simulink model "FeedBack_Linearization"  (R2021b)
(part 8 of 9)

et1504 = ((t3141.*(t8.*(t92-t663)+t15.*(t621-t864))+t2289.*t3617+t2330.*t3620+t2627.*t3444+(t651-t1053).*(t958-t2263+dq7.*t1601+t15.*(t642+t896-t1137-t2220))-t2576.*(t987+t1806+t2261-t3154+t15.*t948)).*(et1333+et1334))./2.0-(t3789.*(et1335+et1336+et1337+et1338+et1339+et1340+et1341+et1342+et1343+et1344))./2.0;
et1505 = t3784.*(t70.*1.8866e-1+t612.*1.8866e-1-t6.*(t88-t617).*5.000000000000001e-5-t13.*(t88-t617).*2.37e-3).*(3.41e+2./1.0e+2);
et1506 = ((t2817+t3324+t3433.*(t614+t13.*(t86-t652))+t2832.*(t639-t1128-t2181+dq5.*t13.*(t86-t652))+t2974.*(t92-t663)+t3422.*(t653-t838)).*(et1345+et1346+et1347+et1348))./2.0-(t3826.*(t609+t846+t847))./2.0+et1349.*et1350-((t3163.*(t8.*(t92-t663)+t15.*(t621-t864))-t1697.*t3336-t2315.*t3618-t2576.*t3437+t2627.*(t933+t1888+t2483+t8.*(t932+t942+t2215+t7.*(t882-t2179)))+t3619.*(t908+t15.*(t921+t14.*(t86-t652)))).*(et1351+et1352))./2.0+(t3060.*(et1353+et1354+et1355+et1356))./2.0-((t859-t1791+t1066.*(t86-t652)).*(et1357+et1358+et1359))./2.0;
et1507 = t3798.*(et1360+et1361+et1362).*(-3.5432e-1)+et1363.*et1364+t3776.*(et1365+et1366).*3.38795-((t3429.*(t1386+t7.*(t88-t617))-t1207.*t3159+t2315.*t3312-(t908+t15.*(t921+t14.*(t86-t652))).*(t884+t1578-t2180+t14.*(t639-t1128-t2181+dq5.*t13.*(t86-t652)))-t1697.*(t631-t885+t1132-t2224)+t2074.*(t926+t988+t1886+t2207+t15.*(-t928+t984+t992+t2187+t2240))).*(et1367+et1368))./2.0;
et1508 = t3674.*(t235+t349+t456+t457+t512+t697.*4.9e-4-t705.*2.019e-2+t1213.*4.9e-4-t1219.*2.019e-2+t1667+t1702+t1710+t1718+t1720+t2072+t2111+t2125).*3.38795;
et1509 = et1369.*et1370-((t6.*(t88-t617).*(t653-t838)-t6.*t831.*(t614+t13.*(t86-t652))+t6.*t573.*(t92-t663)).*(et1371+et1372+et1373))./2.0+et1374.*et1375+(t3824.*(t604.*t815-t572.*(t86-t652)+t10.*t11.*t606))./2.0+(et1376+et1377).*(et1378+et1379+et1380).*3.5432e-1-(t3060.*(et1381+et1382+et1383+et1384+et1385))./2.0+(t3839.*(et1386+et1387+et1388+et1389+et1390))./2.0-((t2735.*(t1529+t15.*(t92-t663))-t1700.*t3618-t1776.*t3619-t2601.*t3161+t3336.*(t648-t657)+t2654.*(t927-t935-t2183+t2206+dq6.*t14.*(t86-t652))).*(et1391+et1392))./2.0+(t3828.*(et1393+et1394+et1395+et1396+et1397))./2.0;
et1510 = (t3840.*(t2074.*(t921+t14.*(t86-t652))+t1738.*(t1386+t7.*(t88-t617))+t1024.*t1207))./2.0-(t3610.*(et1398+et1399+et1400+et1401+et1402+et1403+et1404+et1405+et1406+et1407+et1408))./2.0+(t3610.*(et1409+et1410+et1411+et1412+et1413+et1414+et1415+et1416+et1417))./2.0-(t3666.*(et1418+et1419+et1420))./2.0+((t606.*t827+t815.*t1206-t1295.*(t86-t652)).*(et1421+et1422+et1423))./2.0+et1424.*et1425+(t3842.*(t13.*t831.*t2035+t13.*t573.*(t621-t864)-t13.*t2000.*(t88-t617)))./2.0-t3823.*(et1426+et1427).*3.38795;
et1511 = ((t3140+t3489+t3720+t2832.*(t884+t1578-t2180+t14.*(t639-t1128-t2181+dq5.*t13.*(t86-t652)))+t3436.*(t92-t663)+t3685.*(t653-t838)).*(et1428+et1429+et1430+et1431+et1432))./2.0-t3821.*(et1433+et1434).*3.5432e-1-((-t2961+t3358+t3312.*(t653-t838)).*(et1435+et1436+et1437+et1438+et1439+et1440+et1441+et1442+et1443))./2.0-(t3782.*(et1444+et1445+et1446+et1447+et1448+et1449+et1450+et1451+et1452))./2.0+(t3192.*(et1453+et1454+et1455+et1456+et1457))./2.0;
et1512 = ((t1700.*t2816+t1776.*t2832-(t614+t13.*(t86-t652)).*(t927-t935-t2183+t2206+dq6.*t14.*(t86-t652))-t2735.*(t92-t663)-t2196.*(t648-t657)+t3161.*(t653-t838)).*(et1458+et1459))./2.0-((t3377+t2074.*(t878-t1582+t2184+t7.*(t639-t1128-t2181+dq5.*t13.*(t86-t652)))+t1207.*(t642+t896-t1137-t2220)).*(et1460+et1461+et1462+et1463+et1464+et1465+et1466+et1467+et1468))./2.0;
et1513 = (t2601.*(t853+t983+t2264+t2503)+t2330.*(t884+t1578-t2180+t14.*(t639-t1128-t2181+dq5.*t13.*(t86-t652)))+t2289.*t3312+t2654.*t3168+(t1529+t15.*(t92-t663)).*(t673+t692-t1123-t1805)+(t651-t1053).*(t631-t885+t1132-t2224)).*(et1469+et1470).*(-1.0./2.0)+(t3782.*(et1471+et1472+et1473+et1474+et1475+et1476+et1477+et1478+et1479+et1480))./2.0;
et1514 = t3679.*(t30.*2.0e-4+t33.*5.267999999999999e-2-t82.*5.267999999999999e-2+t89.*2.0e-4).*2.61155;
et1515 = t3780.*(t70.*5.267999999999999e-2+t88.*2.0e-4+t612.*5.267999999999999e-2-t617.*2.0e-4).*(-2.61155);
et1516 = t3781.*(t79.*2.0e-4+t86.*5.267999999999999e-2-t652.*5.267999999999999e-2+t660.*2.0e-4).*(-2.61155);
et1517 = (t1843+t2621+t2648+t606.*t2165+t815.*t2828-(t86-t652).*(t639-t1128-t2181+dq5.*t13.*(t86-t652))).*(et1481+et1482).*(-1.0./2.0)+((t3502+t3544-t3547+t2972.*(t621-t864)+t2196.*(t642+t896-t1137-t2220)+t2816.*(t1487+t2219-t2864+dq6.*t7.*(t88-t617))).*(et1483+et1484+et1485+et1486+et1487))./2.0+et1488.*et1489;
et1518 = -t3291+t3365.*2.900000000000001e-4+t3527+t3642+t3654-t3662-t3665+t2654.*(t884+t1578-t2180+t14.*(t639-t1128-t2181+dq5.*t13.*(t86-t652))).*2.9e-4;
et1519 = t3336.*(t8.*(t92-t663)+t15.*(t621-t864)).*2.94e-3;
et1520 = t2942+t3260+t3261-t1295.*(t878-t1582+t2184+t7.*(t639-t1128-t2181+dq5.*t13.*(t86-t652))).*5.0e-5+t1625.*(t1386+t7.*(t88-t617)).*3.0e-5;
et1521 = t2861.*(t614+t13.*(t86-t652)).*(-1.000000000000001e-3)+t2823.*(t1386+t7.*(t88-t617)).*3.0e-5;
et1522 = t994.*t1207.*3.0e-5+t7.*t3171-t7.*t3358.*3.0e-5+t7.*t3388;
et1523 = t1207.*t2262.*3.0e-5-t1661.*t2074.*3.0e-5;
et1524 = t2074.*t2857.*(-3.0e-5)-t2266.*(t92-t663).*1.000000000000001e-3;
et1525 = t2825.*(t653-t838).*(-1.000000000000001e-3)+t827.*(t642+t896-t1137-t2220).*5.0e-5;
et1526 = t1206.*(t1487+t2219-t2864+dq6.*t7.*(t88-t617)).*5.0e-5+dq6.*t7.*t876.*5.000000000000004e-4;
et1527 = dq6.*t7.*t1462.*5.000000000000004e-4+dq6.*t7.*t1574.*5.000000000000004e-4;
et1528 = -t3294+t3365.*7.950000000000001e-3+t3528+t3648+t3658-t3660-t3663+t2654.*(t884+t1578-t2180+t14.*(t639-t1128-t2181+dq5.*t13.*(t86-t652))).*2.2e-4;
et1529 = t3336.*(t8.*(t92-t663)+t15.*(t621-t864)).*2.900000000000001e-4;
et1530 = t1516.*2.324e-2+t1528.*3.466000000000001e-2+t1668.*2.324e-2+t14.*(t614+t13.*(t86-t652)).*1.9738e-1;
et1531 = t7.*t8.*(t614+t13.*(t86-t652)).*(-3.466000000000001e-2);
et1532 = t2363.*(t1386+t7.*(t88-t617)).*(-7.950000000000001e-3)+t1779.*(t8.*(t92-t663)+t15.*(t621-t864)).*2.900000000000001e-4;
et1533 = t1207.*t1811.*(-7.950000000000001e-3)+t2074.*t2380.*7.950000000000001e-3;
et1534 = t2352.*t2576.*(-2.900000000000001e-4)-t2374.*t2627.*2.900000000000001e-4;
et1535 = t14.*t2654.*(t614+t13.*(t86-t652)).*2.2e-4+t14.*(t1529+t15.*(t92-t663)).*(t92-t663).*2.2e-4;
et1536 = t14.*t2601.*(t653-t838).*2.2e-4;
et1537 = t2675-t2795+t2930+t2939+t3172+t2832.*(t614+t13.*(t86-t652)).*8.933272432898321e-20+t831.*(t639-t1128-t2181+dq5.*t13.*(t86-t652)).*1.0e-5;
et1538 = t2196.*(t92-t663).*8.933272432898321e-20+t2816.*(t653-t838).*8.933272432898321e-20;
et1539 = t2374.*(t884+t1578-t2180+t14.*(t639-t1128-t2181+dq5.*t13.*(t86-t652))).*1.089e-2+t2507.*(t1529+t15.*(t92-t663)).*1.089e-2;
et1540 = t3481.*(t1386+t7.*(t88-t617)).*(-2.2e-4)-t3201.*(t8.*(t92-t663)+t15.*(t621-t864)).*2.9e-4;
et1541 = t1207.*t3202.*(-2.2e-4)+t1811.*t3336.*2.9e-4;
et1542 = t2074.*t3491.*2.2e-4+t2601.*t3035.*1.089e-2;
et1543 = t2352.*t3312.*1.089e-2+t2654.*t3042.*1.089e-2;
et1544 = t2363.*t3618.*2.9e-4+t2380.*t3619.*2.9e-4;
et1545 = t2576.*t3480.*2.9e-4+t2627.*(t1579+t3047+t15.*(t639-t1128-t2181+dq5.*t13.*(t86-t652))+t7.*t1662).*2.9e-4;
et1546 = t1779.*(t631-t885+t1132-t2224).*(-1.089e-2)-t14.*(t92-t663).*(t958-t2263+dq7.*t1601+t15.*(t642+t896-t1137-t2220)).*2.2e-4;
et1547 = t14.*t3620.*(t614+t13.*(t86-t652)).*2.2e-4+t14.*t3617.*(t653-t838).*2.2e-4;
et1548 = t2246-t2269-t3020+t3047.*3.466000000000001e-2-t3048.*2.324e-2+t8.*(t639-t1128-t2181+dq5.*t13.*(t86-t652)).*2.324e-2;
et1549 = t15.*(t639-t1128-t2181+dq5.*t13.*(t86-t652)).*3.466000000000001e-2+t7.*t1662.*3.466000000000001e-2+dq6.*t7.*(t614+t13.*(t86-t652)).*1.9738e-1;
et1550 = dq7.*t7.*t8.*(t614+t13.*(t86-t652)).*2.324e-2;
et1551 = t2925+t3255+t1295.*(t878-t1582+t2184+t7.*(t639-t1128-t2181+dq5.*t13.*(t86-t652))).*4.000000000000028e-5+t1625.*(t1386+t7.*(t88-t617)).*2.32e-3;
et1552 = t2861.*(t614+t13.*(t86-t652)).*(-6.000000000000001e-5)+t2823.*(t1386+t7.*(t88-t617)).*2.32e-3;
et1553 = t2035.*(t639-t1128-t2181+dq5.*t13.*(t86-t652)).*4.000000000000028e-5+t994.*t1207.*2.32e-3;
et1554 = t7.*t2961.*2.32e-3-t7.*t3358.*2.32e-3;
et1555 = t1207.*t2262.*2.32e-3-t1661.*t2074.*2.32e-3;
et1556 = t2074.*t2857.*(-2.32e-3)-t2266.*(t92-t663).*6.000000000000001e-5;
et1557 = t2825.*(t653-t838).*(-6.000000000000001e-5)-t827.*(t642+t896-t1137-t2220).*4.000000000000028e-5;
et1558 = t1206.*(t1487+t2219-t2864+dq6.*t7.*(t88-t617)).*(-4.000000000000028e-5)+dq6.*t7.*t876.*3.0e-5;
et1559 = dq6.*t7.*t1462.*3.0e-5+dq6.*t7.*t1574.*3.0e-5;
et1560 = t7.*t3312.*(t653-t838).*(-2.32e-3);
et1561 = t2374.*(t884+t1578-t2180+t14.*(t639-t1128-t2181+dq5.*t13.*(t86-t652))).*2.9e-4+t2507.*(t1529+t15.*(t92-t663)).*2.9e-4;
et1562 = t3481.*(t1386+t7.*(t88-t617)).*(-2.900000000000001e-4)-t3201.*(t8.*(t92-t663)+t15.*(t621-t864)).*2.94e-3;
et1563 = t1207.*t3202.*(-2.900000000000001e-4)+t1811.*t3336.*2.94e-3;
et1564 = t2074.*t3491.*2.900000000000001e-4+t2601.*t3035.*2.9e-4;
et1565 = t2352.*t3312.*2.9e-4+t2654.*t3042.*2.9e-4;
et1566 = t2363.*t3618.*2.94e-3+t2380.*t3619.*2.94e-3;
et1567 = t2576.*t3480.*2.94e-3+t2627.*(t1579+t3047+t15.*(t639-t1128-t2181+dq5.*t13.*(t86-t652))+t7.*t1662).*2.94e-3;
et1568 = t1779.*(t631-t885+t1132-t2224).*(-2.9e-4)-t14.*(t92-t663).*(t958-t2263+dq7.*t1601+t15.*(t642+t896-t1137-t2220)).*2.900000000000001e-4;
et1569 = t14.*t3620.*(t614+t13.*(t86-t652)).*2.900000000000001e-4+t14.*t3617.*(t653-t838).*2.900000000000001e-4;
et1570 = t2380.*(t884+t1578-t2180+t14.*(t639-t1128-t2181+dq5.*t13.*(t86-t652))).*7.950000000000001e-3+t2266.*(t1529+t15.*(t92-t663)).*2.2e-4;
et1571 = t3483.*(t1386+t7.*(t88-t617)).*(-7.950000000000001e-3)-t3203.*(t8.*(t92-t663)+t15.*(t621-t864)).*2.900000000000001e-4;
et1572 = t1207.*t3204.*(-7.950000000000001e-3)+t2601.*t2825.*2.2e-4;
et1573 = t2654.*t2861.*2.2e-4+t2074.*t3492.*7.950000000000001e-3;
et1574 = t2363.*t3312.*7.950000000000001e-3+t2352.*t3617.*2.900000000000001e-4;
et1575 = t2374.*t3620.*2.900000000000001e-4+t2576.*t3482.*2.900000000000001e-4;
et1576 = t1779.*(t958-t2263+dq7.*t1601+t15.*(t642+t896-t1137-t2220)).*(-2.900000000000001e-4)-t1811.*(t631-t885+t1132-t2224).*7.950000000000001e-3;
et1577 = t2627.*(t1579+t2883+t15.*(t639-t1128-t2181+dq5.*t13.*(t86-t652))+t7.*t1662+t8.*t1661).*2.900000000000001e-4+t14.*t3619.*(t614+t13.*(t86-t652)).*2.2e-4;
et1578 = t14.*t3336.*(t92-t663).*2.2e-4+t14.*t3618.*(t653-t838).*2.2e-4;
et1579 = dq6.*t7.*(t1529+t15.*(t92-t663)).*(t92-t663).*(-2.2e-4)-dq6.*t7.*t2601.*(t653-t838).*2.2e-4;
et1580 = dq6.*t7.*t2654.*(t614+t13.*(t86-t652)).*(-2.2e-4);
et1581 = t2781+t2953.*9.999999999999998e-6+t3142+t2147.*(t614+t13.*(t86-t652)).*4.466636216449161e-20;
et1582 = t2832.*(t614+t13.*(t86-t652)).*1.2e-4+t1295.*(t639-t1128-t2181+dq5.*t13.*(t86-t652)).*1.2e-4;
et1583 = t827.*t2165.*1.2e-4+t1206.*t2828.*1.2e-4;
et1584 = t1070.*(t92-t663).*4.466636216449161e-20+t2196.*(t92-t663).*1.2e-4;
et1585 = t2163.*(t653-t838).*(-4.466636216449161e-20)+t2816.*(t653-t838).*1.2e-4;
et1586 = t876.*1.2e-4+t1462.*1.2e-4;
et1587 = t1574.*1.2e-4-t573.*t827.*9.999999999999998e-6;
et1588 = t831.*t1295.*9.999999999999998e-6-t1206.*(t88-t617).*9.999999999999998e-6;
et1589 = t2380.*(t884+t1578-t2180+t14.*(t639-t1128-t2181+dq5.*t13.*(t86-t652))).*2.2e-4+t2266.*(t1529+t15.*(t92-t663)).*1.089e-2;
et1590 = t3483.*(t1386+t7.*(t88-t617)).*(-2.2e-4)-t3203.*(t8.*(t92-t663)+t15.*(t621-t864)).*2.9e-4;
et1591 = t1207.*t3204.*(-2.2e-4)+t2601.*t2825.*1.089e-2;
et1592 = t2654.*t2861.*1.089e-2+t2074.*t3492.*2.2e-4;
et1593 = t2363.*t3312.*2.2e-4+t2352.*t3617.*2.9e-4;
et1594 = t2374.*t3620.*2.9e-4+t2576.*t3482.*2.9e-4;
et1595 = t1779.*(t958-t2263+dq7.*t1601+t15.*(t642+t896-t1137-t2220)).*(-2.9e-4)-t1811.*(t631-t885+t1132-t2224).*2.2e-4;
et1596 = t2627.*(t1579+t2883+t15.*(t639-t1128-t2181+dq5.*t13.*(t86-t652))+t7.*t1662+t8.*t1661).*2.9e-4+t14.*t3619.*(t614+t13.*(t86-t652)).*1.089e-2;
et1597 = t14.*t3336.*(t92-t663).*1.089e-2+t14.*t3618.*(t653-t838).*1.089e-2;
et1598 = dq6.*t7.*(t1529+t15.*(t92-t663)).*(t92-t663).*(-1.089e-2)-dq6.*t7.*t2601.*(t653-t838).*1.089e-2;
et1599 = dq6.*t7.*t2654.*(t614+t13.*(t86-t652)).*(-1.089e-2);
et1600 = t2925+t3255-t1295.*(t884+t1578-t2180+t14.*(t639-t1128-t2181+dq5.*t13.*(t86-t652))).*3.0e-5+t2857.*(t614+t13.*(t86-t652)).*4.000000000000028e-5;
et1601 = t3042.*(t614+t13.*(t86-t652)).*(-3.0e-5)+t3038.*(t1386+t7.*(t88-t617)).*2.32e-3;
et1602 = t2035.*(t639-t1128-t2181+dq5.*t13.*(t86-t652)).*4.000000000000028e-5+t14.*t2960.*2.32e-3;
et1603 = t14.*t3356.*2.32e-3-t14.*t3357.*2.32e-3;
et1604 = t1207.*t2521.*2.32e-3-t1206.*t3312.*3.0e-5;
et1605 = t2074.*t3045.*(-2.32e-3)+t2262.*(t92-t663).*4.000000000000028e-5;
et1606 = t2507.*(t92-t663).*(-3.0e-5)+t2823.*(t653-t838).*4.000000000000028e-5;
et1607 = t3035.*(t653-t838).*(-3.0e-5)+t827.*(t631-t885+t1132-t2224).*3.0e-5;
et1608 = t2765+t2818-t2907+t3067+t3215+t3235-t3238-t3246+t3268-t3273+t3375+t3551-t3555+t3433.*(t614+t13.*(t86-t652)).*1.2e-4+t2147.*(t639-t1128-t2181+dq5.*t13.*(t86-t652)).*4.466636216449161e-20;
et1609 = t2832.*(t639-t1128-t2181+dq5.*t13.*(t86-t652)).*1.2e-4+t2974.*(t92-t663).*1.2e-4;
et1610 = t3422.*(t653-t838).*1.2e-4;
et1611 = t2363.*(t1386+t7.*(t88-t617)).*(-2.900000000000001e-4)+t1779.*(t8.*(t92-t663)+t15.*(t621-t864)).*2.94e-3;
et1612 = t1207.*t1811.*(-2.900000000000001e-4)+t2074.*t2380.*2.900000000000001e-4;
et1613 = t2352.*t2576.*(-2.94e-3)-t2374.*t2627.*2.94e-3;
et1614 = t14.*t2654.*(t614+t13.*(t86-t652)).*2.9e-4+t14.*(t1529+t15.*(t92-t663)).*(t92-t663).*2.9e-4;
et1615 = t14.*t2601.*(t653-t838).*2.9e-4;
et1616 = t876.*4.466636216449161e-20+t1462.*4.466636216449161e-20+t1574.*4.466636216449161e-20;
et1617 = t573.*t827.*1.0e-5-t831.*t1295.*1.0e-5;
et1618 = t1206.*(t88-t617).*1.0e-5;
et1619 = t2380.*(t884+t1578-t2180+t14.*(t639-t1128-t2181+dq5.*t13.*(t86-t652))).*2.900000000000001e-4+t2266.*(t1529+t15.*(t92-t663)).*2.9e-4;
et1620 = t3483.*(t1386+t7.*(t88-t617)).*(-2.900000000000001e-4)-t3203.*(t8.*(t92-t663)+t15.*(t621-t864)).*2.94e-3;
et1621 = t1207.*t3204.*(-2.900000000000001e-4)+t2601.*t2825.*2.9e-4;
et1622 = t2654.*t2861.*2.9e-4+t2074.*t3492.*2.900000000000001e-4;
et1623 = t2363.*t3312.*2.900000000000001e-4+t2352.*t3617.*2.94e-3;
et1624 = t2374.*t3620.*2.94e-3+t2576.*t3482.*2.94e-3;
et1625 = t1779.*(t958-t2263+dq7.*t1601+t15.*(t642+t896-t1137-t2220)).*(-2.94e-3)-t1811.*(t631-t885+t1132-t2224).*2.900000000000001e-4;
et1626 = t2627.*(t1579+t2883+t15.*(t639-t1128-t2181+dq5.*t13.*(t86-t652))+t7.*t1662+t8.*t1661).*2.94e-3+t14.*t3619.*(t614+t13.*(t86-t652)).*2.9e-4;
et1627 = t14.*t3336.*(t92-t663).*2.9e-4+t14.*t3618.*(t653-t838).*2.9e-4;
et1628 = dq6.*t7.*(t1529+t15.*(t92-t663)).*(t92-t663).*(-2.9e-4)-dq6.*t7.*t2601.*(t653-t838).*2.9e-4;
et1629 = dq6.*t7.*t2654.*(t614+t13.*(t86-t652)).*(-2.9e-4);
et1630 = -t3289+t3365.*2.2e-4+t3526+t3644+t3655-t3661-t3664+t2654.*(t884+t1578-t2180+t14.*(t639-t1128-t2181+dq5.*t13.*(t86-t652))).*1.089e-2;
et1631 = t3336.*(t8.*(t92-t663)+t15.*(t621-t864)).*2.9e-4;
et1632 = -t3289+t3365.*2.2e-4+t3526+t3644+t3655-t3661-t3664+t2654.*(t884+t1578-t2180+t14.*(t639-t1128-t2181+dq5.*t13.*(t86-t652))).*1.089e-2;
et1633 = t3336.*(t8.*(t92-t663)+t15.*(t621-t864)).*2.9e-4;
et1634 = t14.*t876.*3.0e-5+t14.*t1462.*3.0e-5;
et1635 = t14.*t1574.*3.0e-5+t1206.*t2000.*4.000000000000028e-5;
et1636 = t1295.*t2035.*4.000000000000028e-5-t827.*(t621-t864).*4.000000000000028e-5;
et1637 = t7.*t2074.*(t614+t13.*(t86-t652)).*2.32e-3-t7.*(t1386+t7.*(t88-t617)).*(t653-t838).*2.32e-3;
et1638 = t7.*t1207.*(t92-t663).*(-2.32e-3);
et1639 = -t3196-t3253-t3262+t3406+t3452+t2074.*(t878-t1582+t2184+t7.*(t639-t1128-t2181+dq5.*t13.*(t86-t652))).*3.0e-5+t2196.*(t621-t864).*5.0e-5;
et1640 = t3312.*(t653-t838).*5.000000000000004e-4+t1207.*(t642+t896-t1137-t2220).*3.0e-5;
et1641 = -t3291+t3365.*2.900000000000001e-4+t3527+t3642+t3654-t3662-t3665+t2654.*(t884+t1578-t2180+t14.*(t639-t1128-t2181+dq5.*t13.*(t86-t652))).*2.9e-4;
et1642 = t3336.*(t8.*(t92-t663)+t15.*(t621-t864)).*2.94e-3;
et1643 = t2945+t3263+t1295.*(t878-t1582+t2184+t7.*(t639-t1128-t2181+dq5.*t13.*(t86-t652))).*2.81e-3+t1625.*(t1386+t7.*(t88-t617)).*4.000000000000028e-5;
et1644 = t2861.*(t614+t13.*(t86-t652)).*1.0e-4+t2823.*(t1386+t7.*(t88-t617)).*4.000000000000028e-5;
et1645 = t2035.*(t639-t1128-t2181+dq5.*t13.*(t86-t652)).*2.81e-3+t994.*t1207.*4.000000000000028e-5;
et1646 = t7.*t2961.*4.000000000000028e-5-t7.*t3358.*4.000000000000028e-5;
et1647 = t1207.*t2262.*4.000000000000028e-5-t1661.*t2074.*4.000000000000028e-5;
et1648 = t2074.*t2857.*(-4.000000000000028e-5)+t2266.*(t92-t663).*1.0e-4;
et1649 = t2825.*(t653-t838).*1.0e-4-t827.*(t642+t896-t1137-t2220).*2.81e-3;
et1650 = t1206.*(t1487+t2219-t2864+dq6.*t7.*(t88-t617)).*(-2.81e-3)-dq6.*t7.*t876.*5.0e-5;
et1651 = dq6.*t7.*t1462.*(-5.0e-5)-dq6.*t7.*t1574.*5.0e-5;
et1652 = t7.*t3312.*(t653-t838).*(-4.000000000000028e-5);
et1653 = t14.*t876.*5.000000000000004e-4+t14.*t1462.*5.000000000000004e-4;
et1654 = t14.*t1574.*5.000000000000004e-4-t1206.*t2000.*5.0e-5;
et1655 = t1295.*t2035.*(-5.0e-5)+t827.*(t621-t864).*5.0e-5;
et1656 = t7.*t2074.*(t614+t13.*(t86-t652)).*3.0e-5-t7.*(t1386+t7.*(t88-t617)).*(t653-t838).*3.0e-5;
C = ft_11({dq5,dq6,dq7,et1138,et1139,et1140,et1141,et1142,et1143,et1144,et1145,et1146,et1147,et1148,et1149,et1150,et1151,et1152,et1153,et1154,et1155,et1156,et1157,et1158,et1159,et1160,et1161,et1162,et1163,et1164,et1165,et1166,et1167,et1168,et1490,et1491,et1492,et1493,et1494,et1495,et1496,et1497,et1498,et1499,et1500,et1501,et1502,et1503,et1504,et1505,et1506,et1507,et1508,et1509,et1510,et1511,et1512,et1513,et1514,et1515,et1516,et1517,et1518,et1519,et1520,et1521,et1522,et1523,et1524,et1525,et1526,et1527,et1528,et1529,et1530,et1531,et1532,et1533,et1534,et1535,et1536,et1537,et1538,et1539,et1540,et1541,et1542,et1543,et1544,et1545,et1546,et1547,et1548,et1549,et1550,et1551,et1552,et1553,et1554,et1555,et1556,et1557,et1558,et1559,et1560,et1561,et1562,et1563,et1564,et1565,et1566,et1567,et1568,et1569,et1570,et1571,et1572,et1573,et1574,et1575,et1576,et1577,et1578,et1579,et1580,et1581,et1582,et1583,et1584,et1585,et1586,et1587,et1588,et1589,et1590,et1591,et1592,et1593,et1594,et1595,et1596,et1597,et1598,et1599,et1600,et1601,et1602,et1603,et1604,et1605,et1606,et1607,et1608,et1609,et1610,et1611,et1612,et1613,et1614,et1615,et1616,et1617,et1618,et1619,et1620,et1621,et1622,et1623,et1624,et1625,et1626,et1627,et1628,et1629,et1630,et1631,et1632,et1633,et1634,et1635,et1636,et1637,et1638,et1639,et1640,et1641,et1642,et1643,et1644,et1645,et1646,et1647,et1648,et1649,et1650,et1651,et1652,et1653,et1654,et1655,et1656,et217,et218,et219,et220,et221,et222,et223,et224,et225,et226,et227,et228,et229,et685,et686,et687,et688,et689,et690,et691,et692,et693,et694,et695,et696,et697,et698,et699,et700,et701,et702,et703,et704,et705,et706,et707,et708,et709,et710,et711,et712,et713,et714,et715,et716,t1001,t1016,t1017,t1018,t1070,t1128,t1132,t1137,t1206,t1207,t1295,t13,t1329,t1374,t1375,t1386,t1387,t14,t1424,t1462,t1487,t1489,t15,t1515,t1526,t1529,t1574,t1578,t1579,t1581,t1582,t1601,t1604,t1616,t1622,t1625,t1633,t1635,t1657,t1658,t1660,t1661,t1662,t1687,t1726,t1772,t1779,t1811,t1846,t1856,t1898,t1902,t1927,t1934,t1962,t1976,t2000,t2035,t2042,t2044,t2046,t2058,t2074,t2080,t2081,t2108,t2109,t2119,t2139,t2147,t2163,t2165,t2173,t2180,t2181,t2184,t2196,t2198,t2203,t221,t2219,t2220,t2224,t2228,t223,t2231,t2246,t2253,t2262,t2263,t2266,t2269,t2300,t2301,t2352,t2359,t236,t2363,t237,t2370,t2374,t2380,t239,t2407,t2447,t2507,t2521,t2558,t2563,t2570,t2571,t2576,t2581,t2587,t2591,t2601,t2602,t2604,t2611,t2614,t2618,t2620,t2627,t2637,t2647,t2651,t2654,t2656,t2663,t2711,t2781,t2783,t2792,t2795,t2801,t2816,t2817,t2823,t2825,t2828,t2832,t2837,t2838,t2839,t2841,t2844,t2857,t2861,t2864,t2883,t2884,t2914,t2922,t2936,t2945,t2946,t2948,t2949,t2950,t2953,t2954,t2956,t2960,t2961,t2972,t2974,t2991,t2996,t2997,t2998,t3008,t3009,t3020,t3031,t3035,t3038,t3039,t3040,t3041,t3042,t3045,t3047,t3052,t3066,t3071,t3075,t3082,t3083,t3085,t3088,t3092,t3112,t3113,t3122,t3126,t3140,t3142,t3143,t3170,t3172,t3175,t3179,t3181,t3190,t3195,t3196,t3201,t3202,t3203,t3204,t3229,t3232,t3253,t3257,t3262,t3263,t3264,t3269,t3272,t3280,t3284,t3288,t3289,t3290,t3291,t3293,t3294,t3295,t3301,t3312,t3315,t3316,t3321,t3324,t3336,t3340,t3356,t3357,t3358,t3359,t3360,t3361,t3362,t3365,t3366,t3369,t3377,t3382,t3384,t3386,t3392,t3395,t3397,t3398,t3400,t3402,t3403,t3406,t3407,t3411,t3413,t3414,t3417,t3418,t3421,t3422,t3424,t3433,t3436,t3452,t3480,t3481,t3482,t3483,t3489,t3491,t3492,t3495,t3498,t3502,t3526,t3527,t3528,t3535,t3536,t3537,t3538,t3540,t3542,t3544,t3547,t3556,t3559,t3610,t3617,t3618,t3619,t3620,t3625,t3626,t3627,t3642,t3643,t3644,t3645,t3646,t3648,t3649,t3651,t3652,t3653,t3654,t3655,t3658,t3660,t3661,t3662,t3663,t3664,t3665,t3685,t3720,t3751,t3779,t3782,t3783,t3784,t3786,t3788,t3789,t3790,t3796,t3798,t3818,t3820,t3821,t3823,t3828,t3829,t3833,t3835,t3838,t3839,t3840,t3841,t3842,t3843,t3844,t3845,t463,t516,t518,t542,t547,t548,t554,t573,t580,t581,t583,t6,t614,t616,t617,t619,t621,t631,t639,t642,t652,t653,t656,t661,t663,t7,t71,t8,t800,t827,t831,t835,t838,t86,t860,t863,t864,t866,t870,t871,t876,t878,t88,t884,t885,t896,t92,t952,t958,t994});
end
function C = ft_11(ct)
dq5 = ct{1};
dq6 = ct{2};
dq7 = ct{3};
et1138 = ct{4};
et1139 = ct{5};
et1140 = ct{6};
et1141 = ct{7};
et1142 = ct{8};
et1143 = ct{9};
et1144 = ct{10};
et1145 = ct{11};
et1146 = ct{12};
et1147 = ct{13};
et1148 = ct{14};
et1149 = ct{15};
et1150 = ct{16};
et1151 = ct{17};
et1152 = ct{18};
et1153 = ct{19};
et1154 = ct{20};
et1155 = ct{21};
et1156 = ct{22};
et1157 = ct{23};
et1158 = ct{24};
et1159 = ct{25};
et1160 = ct{26};
et1161 = ct{27};
et1162 = ct{28};
et1163 = ct{29};
et1164 = ct{30};
et1165 = ct{31};
et1166 = ct{32};
et1167 = ct{33};
et1168 = ct{34};
et1490 = ct{35};
et1491 = ct{36};
et1492 = ct{37};
et1493 = ct{38};
et1494 = ct{39};
et1495 = ct{40};
et1496 = ct{41};
et1497 = ct{42};
et1498 = ct{43};
et1499 = ct{44};
et1500 = ct{45};
et1501 = ct{46};
et1502 = ct{47};
et1503 = ct{48};
et1504 = ct{49};
et1505 = ct{50};
et1506 = ct{51};
et1507 = ct{52};
et1508 = ct{53};
et1509 = ct{54};
et1510 = ct{55};
et1511 = ct{56};
et1512 = ct{57};
et1513 = ct{58};
et1514 = ct{59};
et1515 = ct{60};
et1516 = ct{61};
et1517 = ct{62};
et1518 = ct{63};
et1519 = ct{64};
et1520 = ct{65};
et1521 = ct{66};
et1522 = ct{67};
et1523 = ct{68};
et1524 = ct{69};
et1525 = ct{70};
et1526 = ct{71};
et1527 = ct{72};
et1528 = ct{73};
et1529 = ct{74};
et1530 = ct{75};
et1531 = ct{76};
et1532 = ct{77};
et1533 = ct{78};
et1534 = ct{79};
et1535 = ct{80};
et1536 = ct{81};
et1537 = ct{82};
et1538 = ct{83};
et1539 = ct{84};
et1540 = ct{85};
et1541 = ct{86};
et1542 = ct{87};
et1543 = ct{88};
et1544 = ct{89};
et1545 = ct{90};
et1546 = ct{91};
et1547 = ct{92};
et1548 = ct{93};
et1549 = ct{94};
et1550 = ct{95};
et1551 = ct{96};
et1552 = ct{97};
et1553 = ct{98};
et1554 = ct{99};
et1555 = ct{100};
et1556 = ct{101};
et1557 = ct{102};
et1558 = ct{103};
et1559 = ct{104};
et1560 = ct{105};
et1561 = ct{106};
et1562 = ct{107};
et1563 = ct{108};
et1564 = ct{109};
et1565 = ct{110};
et1566 = ct{111};
et1567 = ct{112};
et1568 = ct{113};
et1569 = ct{114};
et1570 = ct{115};
et1571 = ct{116};
et1572 = ct{117};
et1573 = ct{118};
et1574 = ct{119};
et1575 = ct{120};
et1576 = ct{121};
et1577 = ct{122};
et1578 = ct{123};
et1579 = ct{124};
et1580 = ct{125};
et1581 = ct{126};
et1582 = ct{127};
et1583 = ct{128};
et1584 = ct{129};
et1585 = ct{130};
et1586 = ct{131};
et1587 = ct{132};
et1588 = ct{133};
et1589 = ct{134};
et1590 = ct{135};
et1591 = ct{136};
et1592 = ct{137};
et1593 = ct{138};
et1594 = ct{139};
et1595 = ct{140};
et1596 = ct{141};
et1597 = ct{142};
et1598 = ct{143};
et1599 = ct{144};
et1600 = ct{145};
et1601 = ct{146};
et1602 = ct{147};
et1603 = ct{148};
et1604 = ct{149};
et1605 = ct{150};
et1606 = ct{151};
et1607 = ct{152};
et1608 = ct{153};
et1609 = ct{154};
et1610 = ct{155};
et1611 = ct{156};
et1612 = ct{157};
et1613 = ct{158};
et1614 = ct{159};
et1615 = ct{160};
et1616 = ct{161};
et1617 = ct{162};
et1618 = ct{163};
et1619 = ct{164};
et1620 = ct{165};
et1621 = ct{166};
et1622 = ct{167};
et1623 = ct{168};
et1624 = ct{169};
et1625 = ct{170};
et1626 = ct{171};
et1627 = ct{172};
et1628 = ct{173};
et1629 = ct{174};
et1630 = ct{175};
et1631 = ct{176};
et1632 = ct{177};
et1633 = ct{178};
et1634 = ct{179};
et1635 = ct{180};
et1636 = ct{181};
et1637 = ct{182};
et1638 = ct{183};
et1639 = ct{184};
et1640 = ct{185};
et1641 = ct{186};
et1642 = ct{187};
et1643 = ct{188};
et1644 = ct{189};
et1645 = ct{190};
et1646 = ct{191};
et1647 = ct{192};
et1648 = ct{193};
et1649 = ct{194};
et1650 = ct{195};
et1651 = ct{196};
et1652 = ct{197};
et1653 = ct{198};
et1654 = ct{199};
et1655 = ct{200};
et1656 = ct{201};
et217 = ct{202};
et218 = ct{203};
et219 = ct{204};
et220 = ct{205};
et221 = ct{206};
et222 = ct{207};
et223 = ct{208};
et224 = ct{209};
et225 = ct{210};
et226 = ct{211};
et227 = ct{212};
et228 = ct{213};
et229 = ct{214};
et685 = ct{215};
et686 = ct{216};
et687 = ct{217};
et688 = ct{218};
et689 = ct{219};
et690 = ct{220};
et691 = ct{221};
et692 = ct{222};
et693 = ct{223};
et694 = ct{224};
et695 = ct{225};
et696 = ct{226};
et697 = ct{227};
et698 = ct{228};
et699 = ct{229};
et700 = ct{230};
et701 = ct{231};
et702 = ct{232};
et703 = ct{233};
et704 = ct{234};
et705 = ct{235};
et706 = ct{236};
et707 = ct{237};
et708 = ct{238};
et709 = ct{239};
et710 = ct{240};
et711 = ct{241};
et712 = ct{242};
et713 = ct{243};
et714 = ct{244};
et715 = ct{245};
et716 = ct{246};
t1001 = ct{247};
t1016 = ct{248};
t1017 = ct{249};
t1018 = ct{250};
t1070 = ct{251};
t1128 = ct{252};
t1132 = ct{253};
t1137 = ct{254};
t1206 = ct{255};
t1207 = ct{256};
t1295 = ct{257};
t13 = ct{258};
t1329 = ct{259};
t1374 = ct{260};
t1375 = ct{261};
t1386 = ct{262};
t1387 = ct{263};
t14 = ct{264};
t1424 = ct{265};
t1462 = ct{266};
t1487 = ct{267};
t1489 = ct{268};
t15 = ct{269};
t1515 = ct{270};
t1526 = ct{271};
t1529 = ct{272};
t1574 = ct{273};
t1578 = ct{274};
t1579 = ct{275};
t1581 = ct{276};
t1582 = ct{277};
t1601 = ct{278};
t1604 = ct{279};
t1616 = ct{280};
t1622 = ct{281};
t1625 = ct{282};
t1633 = ct{283};
t1635 = ct{284};
t1657 = ct{285};
t1658 = ct{286};
t1660 = ct{287};
t1661 = ct{288};
t1662 = ct{289};
t1687 = ct{290};
t1726 = ct{291};
t1772 = ct{292};
t1779 = ct{293};
t1811 = ct{294};
t1846 = ct{295};
t1856 = ct{296};
t1898 = ct{297};
t1902 = ct{298};
t1927 = ct{299};
t1934 = ct{300};
t1962 = ct{301};
t1976 = ct{302};
t2000 = ct{303};
t2035 = ct{304};
t2042 = ct{305};
t2044 = ct{306};
t2046 = ct{307};
t2058 = ct{308};
t2074 = ct{309};
t2080 = ct{310};
t2081 = ct{311};
t2108 = ct{312};
t2109 = ct{313};
t2119 = ct{314};
t2139 = ct{315};
t2147 = ct{316};
t2163 = ct{317};
t2165 = ct{318};
t2173 = ct{319};
t2180 = ct{320};
t2181 = ct{321};
t2184 = ct{322};
t2196 = ct{323};
t2198 = ct{324};
t2203 = ct{325};
t221 = ct{326};
t2219 = ct{327};
t2220 = ct{328};
t2224 = ct{329};
t2228 = ct{330};
t223 = ct{331};
t2231 = ct{332};
t2246 = ct{333};
t2253 = ct{334};
t2262 = ct{335};
t2263 = ct{336};
t2266 = ct{337};
t2269 = ct{338};
t2300 = ct{339};
t2301 = ct{340};
t2352 = ct{341};
t2359 = ct{342};
t236 = ct{343};
t2363 = ct{344};
t237 = ct{345};
t2370 = ct{346};
t2374 = ct{347};
t2380 = ct{348};
t239 = ct{349};
t2407 = ct{350};
t2447 = ct{351};
t2507 = ct{352};
t2521 = ct{353};
t2558 = ct{354};
t2563 = ct{355};
t2570 = ct{356};
t2571 = ct{357};
t2576 = ct{358};
t2581 = ct{359};
t2587 = ct{360};
t2591 = ct{361};
t2601 = ct{362};
t2602 = ct{363};
t2604 = ct{364};
t2611 = ct{365};
t2614 = ct{366};
t2618 = ct{367};
t2620 = ct{368};
t2627 = ct{369};
t2637 = ct{370};
t2647 = ct{371};
t2651 = ct{372};
t2654 = ct{373};
t2656 = ct{374};
t2663 = ct{375};
t2711 = ct{376};
t2781 = ct{377};
t2783 = ct{378};
t2792 = ct{379};
t2795 = ct{380};
t2801 = ct{381};
t2816 = ct{382};
t2817 = ct{383};
t2823 = ct{384};
t2825 = ct{385};
t2828 = ct{386};
t2832 = ct{387};
t2837 = ct{388};
t2838 = ct{389};
t2839 = ct{390};
t2841 = ct{391};
t2844 = ct{392};
t2857 = ct{393};
t2861 = ct{394};
t2864 = ct{395};
t2883 = ct{396};
t2884 = ct{397};
t2914 = ct{398};
t2922 = ct{399};
t2936 = ct{400};
t2945 = ct{401};
t2946 = ct{402};
t2948 = ct{403};
t2949 = ct{404};
t2950 = ct{405};
t2953 = ct{406};
t2954 = ct{407};
t2956 = ct{408};
t2960 = ct{409};
t2961 = ct{410};
t2972 = ct{411};
t2974 = ct{412};
t2991 = ct{413};
t2996 = ct{414};
t2997 = ct{415};
t2998 = ct{416};
t3008 = ct{417};
t3009 = ct{418};
t3020 = ct{419};
t3031 = ct{420};
t3035 = ct{421};
t3038 = ct{422};
t3039 = ct{423};
t3040 = ct{424};
t3041 = ct{425};
t3042 = ct{426};
t3045 = ct{427};
t3047 = ct{428};
t3052 = ct{429};
t3066 = ct{430};
t3071 = ct{431};
t3075 = ct{432};
t3082 = ct{433};
t3083 = ct{434};
t3085 = ct{435};
t3088 = ct{436};
t3092 = ct{437};
t3112 = ct{438};
t3113 = ct{439};
t3122 = ct{440};
t3126 = ct{441};
t3140 = ct{442};
t3142 = ct{443};
t3143 = ct{444};
t3170 = ct{445};
t3172 = ct{446};
t3175 = ct{447};
t3179 = ct{448};
t3181 = ct{449};
t3190 = ct{450};
t3195 = ct{451};
t3196 = ct{452};
t3201 = ct{453};
t3202 = ct{454};
t3203 = ct{455};
t3204 = ct{456};
t3229 = ct{457};
t3232 = ct{458};
t3253 = ct{459};
t3257 = ct{460};
t3262 = ct{461};
t3263 = ct{462};
t3264 = ct{463};
t3269 = ct{464};
t3272 = ct{465};
t3280 = ct{466};
t3284 = ct{467};
t3288 = ct{468};
t3289 = ct{469};
t3290 = ct{470};
t3291 = ct{471};
t3293 = ct{472};
t3294 = ct{473};
t3295 = ct{474};
t3301 = ct{475};
t3312 = ct{476};
t3315 = ct{477};
t3316 = ct{478};
t3321 = ct{479};
t3324 = ct{480};
t3336 = ct{481};
t3340 = ct{482};
t3356 = ct{483};
t3357 = ct{484};
t3358 = ct{485};
t3359 = ct{486};
t3360 = ct{487};
t3361 = ct{488};
t3362 = ct{489};
t3365 = ct{490};
t3366 = ct{491};
t3369 = ct{492};
t3377 = ct{493};
t3382 = ct{494};
t3384 = ct{495};
t3386 = ct{496};
t3392 = ct{497};
t3395 = ct{498};
t3397 = ct{499};
t3398 = ct{500};
t3400 = ct{501};
t3402 = ct{502};
t3403 = ct{503};
t3406 = ct{504};
t3407 = ct{505};
t3411 = ct{506};
t3413 = ct{507};
t3414 = ct{508};
t3417 = ct{509};
t3418 = ct{510};
t3421 = ct{511};
t3422 = ct{512};
t3424 = ct{513};
t3433 = ct{514};
t3436 = ct{515};
t3452 = ct{516};
t3480 = ct{517};
t3481 = ct{518};
t3482 = ct{519};
t3483 = ct{520};
t3489 = ct{521};
t3491 = ct{522};
t3492 = ct{523};
t3495 = ct{524};
t3498 = ct{525};
t3502 = ct{526};
t3526 = ct{527};
t3527 = ct{528};
t3528 = ct{529};
t3535 = ct{530};
t3536 = ct{531};
t3537 = ct{532};
t3538 = ct{533};
t3540 = ct{534};
t3542 = ct{535};
t3544 = ct{536};
t3547 = ct{537};
t3556 = ct{538};
t3559 = ct{539};
t3610 = ct{540};
t3617 = ct{541};
t3618 = ct{542};
t3619 = ct{543};
t3620 = ct{544};
t3625 = ct{545};
t3626 = ct{546};
t3627 = ct{547};
t3642 = ct{548};
t3643 = ct{549};
t3644 = ct{550};
t3645 = ct{551};
t3646 = ct{552};
t3648 = ct{553};
t3649 = ct{554};
t3651 = ct{555};
t3652 = ct{556};
t3653 = ct{557};
t3654 = ct{558};
t3655 = ct{559};
t3658 = ct{560};
t3660 = ct{561};
t3661 = ct{562};
t3662 = ct{563};
t3663 = ct{564};
t3664 = ct{565};
t3665 = ct{566};
t3685 = ct{567};
t3720 = ct{568};
t3751 = ct{569};
t3779 = ct{570};
t3782 = ct{571};
t3783 = ct{572};
t3784 = ct{573};
t3786 = ct{574};
t3788 = ct{575};
t3789 = ct{576};
t3790 = ct{577};
t3796 = ct{578};
t3798 = ct{579};
t3818 = ct{580};
t3820 = ct{581};
t3821 = ct{582};
t3823 = ct{583};
t3828 = ct{584};
t3829 = ct{585};
t3833 = ct{586};
t3835 = ct{587};
t3838 = ct{588};
t3839 = ct{589};
t3840 = ct{590};
t3841 = ct{591};
t3842 = ct{592};
t3843 = ct{593};
t3844 = ct{594};
t3845 = ct{595};
t463 = ct{596};
t516 = ct{597};
t518 = ct{598};
t542 = ct{599};
t547 = ct{600};
t548 = ct{601};
t554 = ct{602};
t573 = ct{603};
t580 = ct{604};
t581 = ct{605};
t583 = ct{606};
t6 = ct{607};
t614 = ct{608};
t616 = ct{609};
t617 = ct{610};
t619 = ct{611};
t621 = ct{612};
t631 = ct{613};
t639 = ct{614};
t642 = ct{615};
t652 = ct{616};
t653 = ct{617};
t656 = ct{618};
t661 = ct{619};
t663 = ct{620};
t7 = ct{621};
t71 = ct{622};
t8 = ct{623};
t800 = ct{624};
t827 = ct{625};
t831 = ct{626};
t835 = ct{627};
t838 = ct{628};
t86 = ct{629};
t860 = ct{630};
t863 = ct{631};
t864 = ct{632};
t866 = ct{633};
t870 = ct{634};
t871 = ct{635};
t876 = ct{636};
t878 = ct{637};
t88 = ct{638};
t884 = ct{639};
t885 = ct{640};
t896 = ct{641};
t92 = ct{642};
t952 = ct{643};
t958 = ct{644};
t994 = ct{645};
et1657 = t7.*t1207.*(t92-t663).*(-3.0e-5);
et1658 = t1687.*(-2.324e-2)+t2246-t2269+t2883.*3.466000000000001e-2-t2884.*2.324e-2-t3020;
et1659 = t8.*(t639-t1128-t2181+dq5.*t13.*(t86-t652)).*2.324e-2+t15.*(t639-t1128-t2181+dq5.*t13.*(t86-t652)).*3.466000000000001e-2+t7.*t1662.*3.466000000000001e-2;
et1660 = t8.*t1661.*3.466000000000001e-2+dq6.*t7.*(t614+t13.*(t86-t652)).*1.9738e-1+dq7.*t7.*t8.*(t614+t13.*(t86-t652)).*2.324e-2;
et1661 = t1657.*3.466000000000001e-2+t1658.*3.466000000000001e-2-t1660.*2.324e-2+t2203-t2228+t2837.*3.466000000000001e-2;
et1662 = t2838.*(-2.324e-2)+t2996-t2998+t3008+dq6.*t7.*(t653-t838).*1.9738e-1+dq7.*t7.*t8.*(t653-t838).*2.324e-2;
et1663 = t2374.*(t884+t1578-t2180+t14.*(t639-t1128-t2181+dq5.*t13.*(t86-t652))).*2.2e-4+t2507.*(t1529+t15.*(t92-t663)).*2.2e-4;
et1664 = t3481.*(t1386+t7.*(t88-t617)).*(-7.950000000000001e-3)-t3201.*(t8.*(t92-t663)+t15.*(t621-t864)).*2.900000000000001e-4;
et1665 = t1207.*t3202.*(-7.950000000000001e-3)+t1811.*t3336.*2.900000000000001e-4;
et1666 = t2074.*t3491.*7.950000000000001e-3+t2601.*t3035.*2.2e-4;
et1667 = t2352.*t3312.*2.2e-4+t2654.*t3042.*2.2e-4;
et1668 = t2363.*t3618.*2.900000000000001e-4+t2380.*t3619.*2.900000000000001e-4;
et1669 = t2576.*t3480.*2.900000000000001e-4+t2627.*(t1579+t3047+t15.*(t639-t1128-t2181+dq5.*t13.*(t86-t652))+t7.*t1662).*2.900000000000001e-4;
et1670 = t1779.*(t631-t885+t1132-t2224).*(-2.2e-4)-t14.*(t92-t663).*(t958-t2263+dq7.*t1601+t15.*(t642+t896-t1137-t2220)).*7.950000000000001e-3;
et1671 = t14.*t3620.*(t614+t13.*(t86-t652)).*7.950000000000001e-3+t14.*t3617.*(t653-t838).*7.950000000000001e-3;
et1672 = t1658.*3.466000000000001e-2+t2203-t2228+t2996-t2998+t3008+t3040.*3.466000000000001e-2-t3041.*2.324e-2+dq6.*t7.*(t653-t838).*1.9738e-1;
et1673 = dq7.*t7.*t8.*(t653-t838).*2.324e-2;
et1674 = -t3294+t3365.*7.950000000000001e-3+t3528+t3648+t3658-t3660-t3663+t2654.*(t884+t1578-t2180+t14.*(t639-t1128-t2181+dq5.*t13.*(t86-t652))).*2.2e-4;
et1675 = t3336.*(t8.*(t92-t663)+t15.*(t621-t864)).*2.900000000000001e-4;
et1676 = -t3196-t3253-t3262+t3406+t3452+t2074.*(t878-t1582+t2184+t7.*(t639-t1128-t2181+dq5.*t13.*(t86-t652))).*3.0e-5+t2196.*(t621-t864).*5.0e-5;
et1677 = t3312.*(t653-t838).*5.000000000000004e-4+t1207.*(t642+t896-t1137-t2220).*3.0e-5;
et1678 = t2832.*(t614+t13.*(t86-t652))+t1295.*(t639-t1128-t2181+dq5.*t13.*(t86-t652))+t827.*t2165+t1206.*t2828+t2196.*(t92-t663)+t2816.*(t653-t838);
et1679 = (-t2447-t2783-t2839+t2841+t3126+t3143+t3232+t2165.*(t92-t663).*1.2e-4+t2828.*(t653-t838).*1.2e-4)./2.0;
et1680 = t1846.*(-2.769999999999999e-3)-t2618.*2.769999999999999e-3;
et1681 = t2620.*2.769999999999999e-3+t2792+t2953.*2.769999999999999e-3+t3175;
et1682 = t2832.*(t614+t13.*(t86-t652)).*2.0e-5+t2196.*(t92-t663).*2.0e-5;
et1683 = t2816.*(t653-t838).*2.0e-5;
et1684 = -t2844-t2914-t2922+t3052+t3229-t3264+t3269+t3280-t3284+t3295+t3301+t3369+t3556-t3559+t3433.*(t614+t13.*(t86-t652)).*9.999999999999998e-6;
et1685 = t2832.*(t639-t1128-t2181+dq5.*t13.*(t86-t652)).*9.999999999999998e-6+t2974.*(t92-t663).*9.999999999999998e-6;
et1686 = t3422.*(t653-t838).*9.999999999999998e-6;
et1687 = t14.*t876.*5.0e-5+t14.*t1462.*5.0e-5;
et1688 = t14.*t1574.*5.0e-5-t1206.*t2000.*2.81e-3;
et1689 = t1295.*t2035.*(-2.81e-3)+t827.*(t621-t864).*2.81e-3;
et1690 = t7.*t2074.*(t614+t13.*(t86-t652)).*(-4.000000000000028e-5)+t7.*(t1386+t7.*(t88-t617)).*(t653-t838).*4.000000000000028e-5;
et1691 = t7.*t1207.*(t92-t663).*4.000000000000028e-5;
et1692 = t3823.*(t619.*2.75e-2+t7.*(t614+t13.*(t86-t652)).*4.9e-4-t14.*(t614+t13.*(t86-t652)).*2.019e-2-t6.*(t86-t652).*2.75e-2);
et1693 = 3.38795;
et1694 = t2363.*(t1386+t7.*(t88-t617)).*(-2.2e-4)+t1779.*(t8.*(t92-t663)+t15.*(t621-t864)).*2.9e-4;
et1695 = t1207.*t1811.*(-2.2e-4)+t2074.*t2380.*2.2e-4;
et1696 = t2352.*t2576.*(-2.9e-4)-t2374.*t2627.*2.9e-4;
et1697 = t14.*t2654.*(t614+t13.*(t86-t652)).*1.089e-2+t14.*(t1529+t15.*(t92-t663)).*(t92-t663).*1.089e-2;
et1698 = t14.*t2601.*(t653-t838).*1.089e-2;
et1699 = t1016.*3.466000000000001e-2+t1017.*3.466000000000001e-2-t1018.*2.324e-2+t1902-t1927+t2300.*3.466000000000001e-2;
et1700 = t2301.*(-2.324e-2)+t2591+t2611-t2663+dq6.*t7.*(t92-t663).*1.9738e-1+dq7.*t7.*t8.*(t92-t663).*2.324e-2;
et1701 = t236+t237+t239+t463+t516+t518+t1772+t1962-t1976+t2173-t2614-t2637-t2647+t3009+dq7.*t1601.*2.324e-2+t15.*(t642+t896-t1137-t2220).*2.324e-2+dq7.*t8.*(t92-t663).*3.466000000000001e-2;
et1702 = dq7.*t15.*(t621-t864).*3.466000000000001e-2;
et1703 = t1017.*3.466000000000001e-2+t1902-t1927+t2570.*3.466000000000001e-2-t2571.*2.324e-2+t2591+t2611-t2663+dq6.*t7.*(t92-t663).*1.9738e-1;
et1704 = dq7.*t7.*t8.*(t92-t663).*2.324e-2;
et1705 = t236+t237+t239+t463+t516+t518+t1772+t1962-t1976+t2173-t2614-t2637-t2647+t3009+dq7.*t1601.*2.324e-2+t15.*(t642+t896-t1137-t2220).*2.324e-2+dq7.*t8.*(t92-t663).*3.466000000000001e-2;
et1706 = dq7.*t15.*(t621-t864).*3.466000000000001e-2;
et1707 = -t2711+t2801-t2954+t2956-t3179+t3181+t2165.*(t92-t663).*4.466636216449161e-20+t2816.*(t88-t617).*1.0e-5;
et1708 = t2828.*(t653-t838).*4.466636216449161e-20;
et1709 = -t2795+t3172+t2147.*(t614+t13.*(t86-t652)).*2.840000000000012e-3+t2832.*(t614+t13.*(t86-t652)).*4.466636216449161e-20;
et1710 = t831.*(t639-t1128-t2181+dq5.*t13.*(t86-t652)).*1.0e-5+t1295.*(t639-t1128-t2181+dq5.*t13.*(t86-t652)).*4.466636216449161e-20;
et1711 = t827.*t2165.*4.466636216449161e-20+t1206.*t2828.*4.466636216449161e-20+t1070.*(t92-t663).*2.840000000000012e-3;
et1712 = t2196.*(t92-t663).*4.466636216449161e-20-t2163.*(t653-t838).*2.840000000000012e-3;
et1713 = t2816.*(t653-t838).*4.466636216449161e-20;
et1714 = t661.*2.75e-2+t835.*2.75e-2+t7.*(t653-t838).*4.9e-4-t14.*(t653-t838).*2.019e-2;
et1715 = (t221.*(2.1e+1./5.0e+1)+t223.*(2.1e+1./5.0e+1)-t542+t547+t548-t554+t580+t581+t583+t800+t1424+t1726+t1856+t1898+t1934+t2042+t2198+t2231+t2253+t2558+t2581+t2587+t2602+t2991+t2997+t3066+t3075+t3082+t3495+t3498).*(-3.38795);
et1716 = t2792+t2953.*2.769999999999999e-3+t3175-t2147.*(t614+t13.*(t86-t652)).*1.0e-5;
et1717 = t2832.*(t614+t13.*(t86-t652)).*9.999999999999998e-6+t1295.*(t639-t1128-t2181+dq5.*t13.*(t86-t652)).*9.999999999999998e-6;
et1718 = t827.*t2165.*9.999999999999998e-6+t1206.*t2828.*9.999999999999998e-6;
et1719 = t1070.*(t92-t663).*(-1.0e-5)+t2196.*(t92-t663).*9.999999999999998e-6;
et1720 = t2163.*(t653-t838).*1.0e-5+t2816.*(t653-t838).*9.999999999999998e-6;
et1721 = t1846.*(-9.999999999999998e-6)-t2618.*9.999999999999998e-6;
et1722 = t2620.*9.999999999999998e-6+t2781+t2953.*9.999999999999998e-6+t3142;
et1723 = t2832.*(t614+t13.*(t86-t652)).*2.4e-4+t2196.*(t92-t663).*2.4e-4;
et1724 = t2816.*(t653-t838).*2.4e-4;
et1725 = t866.*2.324e-2+t871.*3.466000000000001e-2+t1001.*2.324e-2+t14.*(t92-t663).*1.9738e-1;
et1726 = t7.*t8.*(t92-t663).*(-3.466000000000001e-2);
et1727 = t1375.*2.324e-2+t1387.*3.466000000000001e-2+t1633.*2.324e-2+t14.*(t653-t838).*1.9738e-1;
et1728 = t7.*t8.*(t653-t838).*(-3.466000000000001e-2);
et1729 = t876.*9.999999999999998e-6+t1462.*9.999999999999998e-6;
et1730 = t1574.*9.999999999999998e-6-t573.*t827.*2.769999999999999e-3;
et1731 = t831.*t1295.*2.769999999999999e-3-t1206.*(t88-t617).*2.769999999999999e-3;
et1732 = t2832.*(t614+t13.*(t86-t652)).*2.0+t2196.*(t92-t663).*2.0+t2816.*(t653-t838).*2.0;
et1733 = (-t2447-t2783-t2839+t2841+t3126+t3143+t3232+t2165.*(t92-t663).*1.2e-4+t2828.*(t653-t838).*1.2e-4).*(-1.0./2.0);
et1734 = t2945+t3263+t1295.*(t884+t1578-t2180+t14.*(t639-t1128-t2181+dq5.*t13.*(t86-t652))).*5.0e-5+t2857.*(t614+t13.*(t86-t652)).*2.81e-3;
et1735 = t3042.*(t614+t13.*(t86-t652)).*5.0e-5+t3038.*(t1386+t7.*(t88-t617)).*4.000000000000028e-5;
et1736 = t2035.*(t639-t1128-t2181+dq5.*t13.*(t86-t652)).*2.81e-3+t14.*t2960.*4.000000000000028e-5;
et1737 = t14.*t3356.*4.000000000000028e-5-t14.*t3357.*4.000000000000028e-5;
et1738 = t1207.*t2521.*4.000000000000028e-5+t1206.*t3312.*5.0e-5;
et1739 = t2074.*t3045.*(-4.000000000000028e-5)+t2262.*(t92-t663).*2.81e-3;
et1740 = t2507.*(t92-t663).*5.0e-5+t2823.*(t653-t838).*2.81e-3;
et1741 = t3035.*(t653-t838).*5.0e-5-t827.*(t631-t885+t1132-t2224).*5.0e-5;
et1742 = t2936+t3257+t1295.*(t884+t1578-t2180+t14.*(t639-t1128-t2181+dq5.*t13.*(t86-t652))).*5.000000000000004e-4+t2857.*(t614+t13.*(t86-t652)).*5.0e-5;
et1743 = t3042.*(t614+t13.*(t86-t652)).*5.000000000000004e-4-t3038.*(t1386+t7.*(t88-t617)).*3.0e-5;
et1744 = t2035.*(t639-t1128-t2181+dq5.*t13.*(t86-t652)).*5.0e-5-t14.*t2960.*3.0e-5;
et1745 = t14.*t3356.*(-3.0e-5)+t14.*t3395-t1207.*t2521.*3.0e-5;
et1746 = t1206.*t3312.*5.000000000000004e-4+t2074.*t3045.*3.0e-5;
et1747 = t2262.*(t92-t663).*5.0e-5+t2507.*(t92-t663).*5.000000000000004e-4;
et1748 = t2823.*(t653-t838).*5.0e-5+t3035.*(t653-t838).*5.000000000000004e-4;
et1749 = t827.*(t631-t885+t1132-t2224).*(-5.000000000000004e-4);
et1750 = t3779.*(t71.*2.37e-3+t92.*5.000000000000001e-5+t656.*2.37e-3-t663.*5.000000000000001e-5).*(-3.41e+2./1.0e+2);
et1751 = t3784.*(t653.*5.000000000000001e-5+t661.*2.37e-3+t835.*2.37e-3-t838.*5.000000000000001e-5).*(-3.41e+2./1.0e+2)-(t3841.*(t14.*t876+t14.*t1462+t14.*t1574))./2.0;
et1752 = ((-t3201.*(t8.*(t92-t663)+t15.*(t621-t864))+t1811.*t3336+t2363.*t3618+t2380.*t3619+t2576.*t3480+t2627.*(t1579+t3047+t15.*(t639-t1128-t2181+dq5.*t13.*(t86-t652))+t7.*t1662)).*(et1518+et1519))./2.0+((-t2961+t3358+t3312.*(t653-t838)).*(et1520+et1521+et1522+et1523+et1524+et1525+et1526+et1527))./2.0-((t3481.*(t1386+t7.*(t88-t617))+t1207.*t3202-t2074.*t3491+t14.*(t92-t663).*(t958-t2263+dq7.*t1601+t15.*(t642+t896-t1137-t2220))-t14.*t3620.*(t614+t13.*(t86-t652))-t14.*t3617.*(t653-t838)).*(et1528+et1529))./2.0+t3835.*(et1530+et1531).*3.5432e-1;
et1753 = (t3788.*(-t2359+t2950+t3272+t831.*(t639-t1128-t2181+dq5.*t13.*(t86-t652))))./2.0-(t3838.*(et1532+et1533+et1534+et1535+et1536))./2.0+(t3272.*(et1537+et1538))./2.0+((-t3113+t3418+t2654.*(t884+t1578-t2180+t14.*(t639-t1128-t2181+dq5.*t13.*(t86-t652)))).*(et1539+et1540+et1541+et1542+et1543+et1544+et1545+et1546+et1547))./2.0-t3798.*(et1548+et1549+et1550).*3.5432e-1+((t3377+t2074.*(t878-t1582+t2184+t7.*(t639-t1128-t2181+dq5.*t13.*(t86-t652)))+t1207.*(t642+t896-t1137-t2220)).*(et1551+et1552+et1553+et1554+et1555+et1556+et1557+et1558+et1559+et1560))./2.0-(t3789.*(et1561+et1562+et1563+et1564+et1565+et1566+et1567+et1568+et1569))./2.0;
et1754 = t3842.*(t1206.*t2000+t1295.*t2035-t827.*(t621-t864)).*(-1.0./2.0)-(t3782.*(et1570+et1571+et1572+et1573+et1574+et1575+et1576+et1577+et1578+et1579+et1580))./2.0+((t3031+t2165.*(t92-t663)+t2828.*(t653-t838)).*(et1581+et1582+et1583+et1584+et1585))./2.0;
et1755 = t3786.*(t614.*5.000000000000001e-5+t619.*2.37e-3-t6.*(t86-t652).*2.37e-3+t13.*(t86-t652).*5.000000000000001e-5).*(3.41e+2./1.0e+2);
et1756 = (et1586+et1587+et1588).*(t2817+t3324+t3433.*(t614+t13.*(t86-t652))+t2832.*(t639-t1128-t2181+dq5.*t13.*(t86-t652))+t2974.*(t92-t663)+t3422.*(t653-t838)).*(-1.0./2.0)-((-t3113+t3418+t2654.*(t884+t1578-t2180+t14.*(t639-t1128-t2181+dq5.*t13.*(t86-t652)))).*(et1589+et1590+et1591+et1592+et1593+et1594+et1595+et1596+et1597+et1598+et1599))./2.0-(t3820.*(t2651+t3083+t2857.*(t614+t13.*(t86-t652))+t2035.*(t639-t1128-t2181+dq5.*t13.*(t86-t652))+t2262.*(t92-t663)+t2823.*(t653-t838)))./2.0;
et1757 = (t3377+t2074.*(t878-t1582+t2184+t7.*(t639-t1128-t2181+dq5.*t13.*(t86-t652)))+t1207.*(t642+t896-t1137-t2220)).*(et1600+et1601+et1602+et1603+et1604+et1605+et1606+et1607).*(-1.0./2.0)-((t876+t1462+t1574).*(et1608+et1609+et1610))./2.0+(t3818.*(t1625.*(t1386+t7.*(t88-t617))+t2823.*(t1386+t7.*(t88-t617))+t994.*t1207+t7.*t2961+t7.*t3340+t7.*t3362+t1207.*t2262+t1622.*t2074-t2074.*t2857))./2.0-(t3839.*(et1611+et1612+et1613+et1614+et1615))./2.0-((et1616+et1617+et1618).*(t2407+t2563+t3085-t3092-t3122+t2147.*(t639-t1128-t2181+dq5.*t13.*(t86-t652))))./2.0+(t3789.*(et1619+et1620+et1621+et1622+et1623+et1624+et1625+et1626+et1627+et1628+et1629))./2.0;
et1758 = (t952.*(t1529+t15.*(t92-t663))+t2266.*(t1529+t15.*(t92-t663))+t1581.*t2601+t1616.*t2654+t2601.*t2825+t2654.*t2861+t14.*t3619.*(t614+t13.*(t86-t652))+t14.*t3336.*(t92-t663)+t14.*t3618.*(t653-t838)).*(et1630+et1631).*(-1.0./2.0)+((t2374.*(t884+t1578-t2180+t14.*(t639-t1128-t2181+dq5.*t13.*(t86-t652)))+t2507.*(t1529+t15.*(t92-t663))+t2601.*t3035+t2352.*t3312+t2654.*t3042-t1779.*(t631-t885+t1132-t2224)).*(et1632+et1633))./2.0-(t3828.*(et1634+et1635+et1636+et1637+et1638))./2.0;
et1759 = (t2861.*(t614+t13.*(t86-t652)).*2.0+t2266.*(t92-t663).*2.0+t2825.*(t653-t838).*2.0-dq6.*t7.*t876-dq6.*t7.*t1462-dq6.*t7.*t1574).*(et1639+et1640).*(-1.0./2.0)+(t3840.*(-t7.*t2074.*(t614+t13.*(t86-t652))+t7.*(t1386+t7.*(t88-t617)).*(t653-t838)+t7.*t1207.*(t92-t663)))./2.0-(t3843.*(t14.*t2654.*(t614+t13.*(t86-t652))+t14.*(t1529+t15.*(t92-t663)).*(t92-t663)+t14.*t2601.*(t653-t838)))./2.0;
et1760 = (-t3203.*(t8.*(t92-t663)+t15.*(t621-t864))+t2352.*t3617+t2374.*t3620+t2576.*t3482-t1779.*(t958-t2263+dq7.*t1601+t15.*(t642+t896-t1137-t2220))+t2627.*(t1579+t2883+t15.*(t639-t1128-t2181+dq5.*t13.*(t86-t652))+t7.*t1662+t8.*t1661)).*(et1641+et1642).*(-1.0./2.0)+(t3610.*(et1643+et1644+et1645+et1646+et1647+et1648+et1649+et1650+et1651+et1652))./2.0+(t3788.*(t2359+t2948+t2953))./2.0-((t3140+t3489+t3720+t2832.*(t884+t1578-t2180+t14.*(t639-t1128-t2181+dq5.*t13.*(t86-t652)))+t3436.*(t92-t663)+t3685.*(t653-t838)).*(et1653+et1654+et1655+et1656+et1657))./2.0+t3798.*(et1658+et1659+et1660).*3.5432e-1;
et1761 = t3796.*(et1661+et1662).*3.5432e-1+(t3782.*(et1663+et1664+et1665+et1666+et1667+et1668+et1669+et1670+et1671))./2.0-t3796.*(et1672+et1673).*3.5432e-1-((t2380.*(t884+t1578-t2180+t14.*(t639-t1128-t2181+dq5.*t13.*(t86-t652)))-t3483.*(t1386+t7.*(t88-t617))-t1207.*t3204+t2074.*t3492+t2363.*t3312-t1811.*(t631-t885+t1132-t2224)).*(et1674+et1675))./2.0;
et1762 = ((t1295.*(t884+t1578-t2180+t14.*(t639-t1128-t2181+dq5.*t13.*(t86-t652)))+t3042.*(t614+t13.*(t86-t652))+t1206.*t3312+t2507.*(t92-t663)+t3035.*(t653-t838)-t827.*(t631-t885+t1132-t2224)).*(et1676+et1677))./2.0+et1678.*et1679+((t2370-t2949+t2816.*(t88-t617)).*(et1680+et1681+et1682+et1683))./2.0+((t573.*t827-t831.*t1295+t1206.*(t88-t617)).*(et1684+et1685+et1686))./2.0+((t3502+t3544-t3547+t2972.*(t621-t864)+t2196.*(t642+t896-t1137-t2220)+t2816.*(t1487+t2219-t2864+dq6.*t7.*(t88-t617))).*(et1687+et1688+et1689+et1690+et1691))./2.0;
et1763 = t3818.*(t3038.*(t1386+t7.*(t88-t617))+t14.*t2960+t14.*t3356+t14.*t3361+t1207.*t2521-t2074.*t3045).*(-1.0./2.0)+et1692.*et1693-(t3829.*(et1694+et1695+et1696+et1697+et1698))./2.0-(et1699+et1700).*(et1701+et1702).*3.5432e-1+(et1703+et1704).*(et1705+et1706).*3.5432e-1+((t2147.*(t614+t13.*(t86-t652))+t1070.*(t92-t663)-t2163.*(t653-t838)).*(et1707+et1708))./2.0;
et1764 = t3790.*(t71.*2.75e-2+t656.*2.75e-2+t7.*(t92-t663).*4.9e-4-t14.*(t92-t663).*2.019e-2).*3.38795;
et1765 = t3272.*(et1709+et1710+et1711+et1712+et1713).*(-1.0./2.0)+et1714.*et1715-((t2370-t2949+t2816.*(t88-t617)).*(et1716+et1717+et1718+et1719+et1720))./2.0-((t3031+t2165.*(t92-t663)+t2828.*(t653-t838)).*(et1721+et1722+et1723+et1724))./2.0-t3821.*(et1725+et1726).*3.5432e-1-t3833.*(et1727+et1728).*3.5432e-1+(t3845.*(t2363.*(t1386+t7.*(t88-t617))+t1207.*t1811-t2074.*t2380))./2.0+(t3844.*(-t1779.*(t8.*(t92-t663)+t15.*(t621-t864))+t2352.*t2576+t2374.*t2627))./2.0+(t3783.*(et1729+et1730+et1731))./2.0;
et1766 = (t3820.*(t2651+t3083+t1295.*(t878-t1582+t2184+t7.*(t639-t1128-t2181+dq5.*t13.*(t86-t652)))+t2035.*(t639-t1128-t2181+dq5.*t13.*(t86-t652))-t827.*(t642+t896-t1137-t2220)-t1206.*(t1487+t2219-t2864+dq6.*t7.*(t88-t617))))./2.0+et1732.*et1733-(t3610.*(et1734+et1735+et1736+et1737+et1738+et1739+et1740+et1741))./2.0+((-t2961+t3358+t3312.*(t653-t838)).*(et1742+et1743+et1744+et1745+et1746+et1747+et1748+et1749))./2.0;
et1767 = -t3289+t3365.*2.2e-4+t3526+t3644+t3655-t3661-t3664+t2654.*(t884+t1578-t2180+t14.*(t639-t1128-t2181+dq5.*t13.*(t86-t652))).*1.089e-2;
et1768 = t3336.*(t8.*(t92-t663)+t15.*(t621-t864)).*2.9e-4;
et1769 = t15.*t1329.*7.950000000000001e-3+t15.*t2058.*7.950000000000001e-3;
et1770 = t15.*t2108.*7.950000000000001e-3+t2000.*t2601.*2.2e-4;
et1771 = t2035.*t2654.*2.2e-4-(t1529+t15.*(t92-t663)).*(t621-t864).*2.2e-4;
et1772 = t8.*t2576.*(t1386+t7.*(t88-t617)).*(-2.900000000000001e-4)+t8.*t1207.*(t8.*(t92-t663)+t15.*(t621-t864)).*2.900000000000001e-4;
et1773 = t8.*t2074.*t2627.*2.900000000000001e-4;
et1774 = t1329.*4.000000000000028e-5+t2058.*4.000000000000028e-5;
et1775 = t2108.*4.000000000000028e-5-t2035.*(t614+t13.*(t86-t652)).*5.0e-5;
et1776 = t2000.*(t653-t838).*(-5.0e-5)+(t92-t663).*(t621-t864).*5.0e-5;
et1777 = t3170+t3392+t3398+t2035.*(t878-t1582+t2184+t7.*(t639-t1128-t2181+dq5.*t13.*(t86-t652))).*2.32e-3;
et1778 = t2074.*(t884+t1578-t2180+t14.*(t639-t1128-t2181+dq5.*t13.*(t86-t652))).*2.32e-3+t2816.*(t1386+t7.*(t88-t617)).*4.000000000000028e-5;
et1779 = t3312.*(t1386+t7.*(t88-t617)).*(-2.32e-3)+t1207.*t2196.*4.000000000000028e-5;
et1780 = t2074.*t2832.*(-4.000000000000028e-5)+t1207.*(t631-t885+t1132-t2224).*2.32e-3;
et1781 = t2000.*(t1487+t2219-t2864+dq6.*t7.*(t88-t617)).*(-2.32e-3)+(t621-t864).*(t642+t896-t1137-t2220).*2.32e-3;
et1782 = t1374.*2.019e-2+t1386.*4.9e-4+t7.*(t88-t617).*4.9e-4-t14.*(t88-t617).*2.019e-2;
et1783 = (t221.*(2.1e+1./5.0e+1)+t223.*(2.1e+1./5.0e+1)-t542+t547+t548-t554+t580+t581+t583+t800+t1424+t1726+t1856+t1898+t1934+t2042+t2198+t2231+t2253+t2558+t2581+t2587+t2602+t2991+t2997+t3066+t3075+t3082+t3495+t3498).*3.38795;
et1784 = t3195+t3402+t3407+t2035.*(t878-t1582+t2184+t7.*(t639-t1128-t2181+dq5.*t13.*(t86-t652))).*3.0e-5;
et1785 = t2074.*(t884+t1578-t2180+t14.*(t639-t1128-t2181+dq5.*t13.*(t86-t652))).*3.0e-5-t2816.*(t1386+t7.*(t88-t617)).*5.0e-5;
et1786 = t3312.*(t1386+t7.*(t88-t617)).*(-3.0e-5)-t1207.*t2196.*5.0e-5;
et1787 = t2074.*t2832.*5.0e-5+t1207.*(t631-t885+t1132-t2224).*3.0e-5;
et1788 = t2000.*(t1487+t2219-t2864+dq6.*t7.*(t88-t617)).*(-3.0e-5)+(t621-t864).*(t642+t896-t1137-t2220).*3.0e-5;
et1789 = t1374.*1.9738e-1+t8.*(t1386+t7.*(t88-t617)).*3.466000000000001e-2-t15.*(t1386+t7.*(t88-t617)).*2.324e-2;
et1790 = t14.*(t88-t617).*(-1.9738e-1);
et1791 = -t3196-t3253-t3262+t3406+t3452+t2074.*(t878-t1582+t2184+t7.*(t639-t1128-t2181+dq5.*t13.*(t86-t652))).*3.0e-5+t2196.*(t621-t864).*5.0e-5;
et1792 = t3312.*(t653-t838).*5.000000000000004e-4+t1207.*(t642+t896-t1137-t2220).*3.0e-5;
et1793 = t3071.*3.0e-5+t3088.*3.0e-5+t3170+t3392+t3398;
et1794 = t2074.*(t884+t1578-t2180+t14.*(t639-t1128-t2181+dq5.*t13.*(t86-t652))).*4.639999999999999e-3-t3312.*(t1386+t7.*(t88-t617)).*4.639999999999999e-3;
et1795 = t2196.*(t621-t864).*(-3.0e-5)+t1207.*(t631-t885+t1132-t2224).*4.639999999999999e-3;
et1796 = t1329.*2.32e-3+t2058.*2.32e-3;
et1797 = t2108.*2.32e-3+t2035.*(t614+t13.*(t86-t652)).*3.0e-5;
et1798 = t2000.*(t653-t838).*3.0e-5-(t92-t663).*(t621-t864).*3.0e-5;
et1799 = t3288+t3535+t3538+t3315.*(t1386+t7.*(t88-t617)).*1.089e-2-t3384.*(t1386+t7.*(t88-t617)).*2.2e-4;
et1800 = t15.*t3360.*(-2.9e-4)+t15.*t3626.*2.9e-4;
et1801 = t1207.*t3039.*(-2.2e-4)-t2074.*t3386.*2.2e-4;
et1802 = t2000.*t3617.*2.2e-4+t2035.*t3620.*2.2e-4;
et1803 = t2576.*t3382.*2.9e-4+(t8.*(t92-t663)+t15.*(t621-t864)).*(t1489+t8.*(t631-t885+t1132-t2224)).*2.9e-4;
et1804 = (t621-t864).*(t958-t2263+dq7.*t1601+t15.*(t642+t896-t1137-t2220)).*2.2e-4;
et1805 = t2627.*(t2139+t8.*(t884+t1578-t2180+t14.*(t639-t1128-t2181+dq5.*t13.*(t86-t652)))).*2.9e-4-t8.*t1207.*(t631-t885+t1132-t2224).*1.089e-2;
et1806 = t8.*t2074.*(t884+t1578-t2180+t14.*(t639-t1128-t2181+dq5.*t13.*(t86-t652))).*(-1.089e-2)-t15.*t3618.*(t1386+t7.*(t88-t617)).*2.9e-4;
et1807 = -t3291+t3365.*2.900000000000001e-4+t3527+t3642+t3654-t3662-t3665+t2654.*(t884+t1578-t2180+t14.*(t639-t1128-t2181+dq5.*t13.*(t86-t652))).*2.9e-4;
et1808 = t3336.*(t8.*(t92-t663)+t15.*(t621-t864)).*2.94e-3;
et1809 = t15.*t1329.*2.900000000000001e-4+t15.*t2058.*2.900000000000001e-4;
et1810 = t15.*t2108.*2.900000000000001e-4+t2000.*t2601.*2.9e-4;
et1811 = t2035.*t2654.*2.9e-4-(t1529+t15.*(t92-t663)).*(t621-t864).*2.9e-4;
et1812 = t8.*t2576.*(t1386+t7.*(t88-t617)).*(-2.94e-3)+t8.*t1207.*(t8.*(t92-t663)+t15.*(t621-t864)).*2.94e-3;
et1813 = t8.*t2074.*t2627.*2.94e-3;
et1814 = t3290+t3536+t3540+t3315.*(t1386+t7.*(t88-t617)).*2.9e-4-t3384.*(t1386+t7.*(t88-t617)).*2.900000000000001e-4;
et1815 = t15.*t3360.*(-2.94e-3)+t15.*t3626.*2.94e-3;
et1816 = t1207.*t3039.*(-2.900000000000001e-4)-t2074.*t3386.*2.900000000000001e-4;
et1817 = t2000.*t3617.*2.900000000000001e-4+t2035.*t3620.*2.900000000000001e-4;
et1818 = t2576.*t3382.*2.94e-3+(t8.*(t92-t663)+t15.*(t621-t864)).*(t1489+t8.*(t631-t885+t1132-t2224)).*2.94e-3;
et1819 = (t621-t864).*(t958-t2263+dq7.*t1601+t15.*(t642+t896-t1137-t2220)).*2.900000000000001e-4;
et1820 = t2627.*(t2139+t8.*(t884+t1578-t2180+t14.*(t639-t1128-t2181+dq5.*t13.*(t86-t652)))).*2.94e-3;
et1821 = t8.*t1207.*(t631-t885+t1132-t2224).*(-2.9e-4)-t8.*t2074.*(t884+t1578-t2180+t14.*(t639-t1128-t2181+dq5.*t13.*(t86-t652))).*2.9e-4;
et1822 = t15.*t3618.*(t1386+t7.*(t88-t617)).*(-2.94e-3);
et1823 = t1329.*3.0e-5+t2058.*3.0e-5;
et1824 = t2108.*3.0e-5+t2035.*(t614+t13.*(t86-t652)).*5.000000000000004e-4;
et1825 = t2000.*(t653-t838).*5.000000000000004e-4-(t92-t663).*(t621-t864).*5.000000000000004e-4;
et1826 = t3071.*5.000000000000004e-4+t3088.*5.000000000000004e-4+t3195+t3402+t3407;
et1827 = t2074.*(t884+t1578-t2180+t14.*(t639-t1128-t2181+dq5.*t13.*(t86-t652))).*6.000000000000001e-5-t3312.*(t1386+t7.*(t88-t617)).*6.000000000000001e-5;
et1828 = t2196.*(t621-t864).*(-5.000000000000004e-4)+t1207.*(t631-t885+t1132-t2224).*6.000000000000001e-5;
et1829 = -t3289+t3365.*2.2e-4+t3526+t3644+t3655-t3661-t3664+t2654.*(t884+t1578-t2180+t14.*(t639-t1128-t2181+dq5.*t13.*(t86-t652))).*1.089e-2;
et1830 = t3336.*(t8.*(t92-t663)+t15.*(t621-t864)).*2.9e-4;
et1831 = -t3190-t3397+t3400+t2035.*(t878-t1582+t2184+t7.*(t639-t1128-t2181+dq5.*t13.*(t86-t652))).*4.000000000000028e-5;
et1832 = t2074.*(t884+t1578-t2180+t14.*(t639-t1128-t2181+dq5.*t13.*(t86-t652))).*4.000000000000028e-5+t2816.*(t1386+t7.*(t88-t617)).*2.81e-3;
et1833 = t3312.*(t1386+t7.*(t88-t617)).*(-4.000000000000028e-5)+t1207.*t2196.*2.81e-3;
et1834 = t2074.*t2832.*(-2.81e-3)+t1207.*(t631-t885+t1132-t2224).*4.000000000000028e-5;
et1835 = t2000.*(t1487+t2219-t2864+dq6.*t7.*(t88-t617)).*(-4.000000000000028e-5)+(t621-t864).*(t642+t896-t1137-t2220).*4.000000000000028e-5;
et1836 = -t3294+t3365.*7.950000000000001e-3+t3528+t3648+t3658-t3660-t3663+t2654.*(t884+t1578-t2180+t14.*(t639-t1128-t2181+dq5.*t13.*(t86-t652))).*2.2e-4;
et1837 = t3336.*(t8.*(t92-t663)+t15.*(t621-t864)).*2.900000000000001e-4;
et1838 = t15.*t1329.*2.2e-4+t15.*t2058.*2.2e-4;
et1839 = t15.*t2108.*2.2e-4+t2000.*t2601.*1.089e-2;
et1840 = t2035.*t2654.*1.089e-2-(t1529+t15.*(t92-t663)).*(t621-t864).*1.089e-2;
et1841 = t8.*t2576.*(t1386+t7.*(t88-t617)).*(-2.9e-4)+t8.*t1207.*(t8.*(t92-t663)+t15.*(t621-t864)).*2.9e-4;
et1842 = t8.*t2074.*t2627.*2.9e-4;
et1843 = -t3294+t3365.*7.950000000000001e-3+t3528+t3648+t3658-t3660-t3663+t2654.*(t884+t1578-t2180+t14.*(t639-t1128-t2181+dq5.*t13.*(t86-t652))).*2.2e-4;
et1844 = t3336.*(t8.*(t92-t663)+t15.*(t621-t864)).*2.900000000000001e-4;
et1845 = t2946+t3190+t3253+t3262+t3397+t3403-t2074.*(t884+t1578-t2180+t14.*(t639-t1128-t2181+dq5.*t13.*(t86-t652))).*8.000000000000056e-5+t3312.*(t1386+t7.*(t88-t617)).*8.000000000000056e-5;
et1846 = t1207.*(t631-t885+t1132-t2224).*(-8.000000000000056e-5);
et1847 = -t3196-t3253-t3262+t3406+t3452+t2074.*(t878-t1582+t2184+t7.*(t639-t1128-t2181+dq5.*t13.*(t86-t652))).*3.0e-5+t2196.*(t621-t864).*5.0e-5;
et1848 = t3312.*(t653-t838).*5.000000000000004e-4+t1207.*(t642+t896-t1137-t2220).*3.0e-5;
et1849 = t3290+t3536+t3540-t3316.*(t1386+t7.*(t88-t617)).*5.800000000000002e-4+t1489.*(t8.*(t92-t663)+t15.*(t621-t864)).*2.94e-3;
et1850 = t8.*t3365.*(-2.94e-3)-t8.*t3627.*2.94e-3;
et1851 = t2139.*t2627.*2.94e-3+t2000.*t3618.*2.9e-4;
et1852 = t2035.*t3619.*2.9e-4+t2576.*t3315.*2.94e-3;
et1853 = t3336.*(t621-t864).*(-2.9e-4)+t8.*(t8.*(t92-t663)+t15.*(t621-t864)).*(t631-t885+t1132-t2224).*2.94e-3;
et1854 = t15.*t1207.*(t631-t885+t1132-t2224).*5.800000000000002e-4+t15.*t2074.*(t884+t1578-t2180+t14.*(t639-t1128-t2181+dq5.*t13.*(t86-t652))).*5.800000000000002e-4;
et1855 = t8.*t2627.*(t884+t1578-t2180+t14.*(t639-t1128-t2181+dq5.*t13.*(t86-t652))).*2.94e-3+t8.*t3617.*(t1386+t7.*(t88-t617)).*2.94e-3;
et1856 = dq7.*t8.*t1329.*(-2.900000000000001e-4)-dq7.*t8.*t2058.*2.900000000000001e-4;
et1857 = dq7.*t8.*t2108.*(-2.900000000000001e-4)-dq7.*t15.*t2576.*(t1386+t7.*(t88-t617)).*2.94e-3;
et1858 = t3293+t3537+t3542+t3315.*(t1386+t7.*(t88-t617)).*2.2e-4-t3384.*(t1386+t7.*(t88-t617)).*7.950000000000001e-3;
et1859 = t15.*t3360.*(-2.900000000000001e-4)+t15.*t3643+t15.*t3651-t1207.*t3039.*7.950000000000001e-3;
et1860 = t2074.*t3386.*(-7.950000000000001e-3)+t2000.*t3617.*7.950000000000001e-3;
et1861 = t2035.*t3620.*7.950000000000001e-3+t2576.*t3382.*2.900000000000001e-4;
et1862 = (t8.*(t92-t663)+t15.*(t621-t864)).*(t1489+t8.*(t631-t885+t1132-t2224)).*2.900000000000001e-4;
et1863 = (t621-t864).*(t958-t2263+dq7.*t1601+t15.*(t642+t896-t1137-t2220)).*7.950000000000001e-3;
et1864 = t2627.*(t2139+t8.*(t884+t1578-t2180+t14.*(t639-t1128-t2181+dq5.*t13.*(t86-t652)))).*2.900000000000001e-4-t8.*t1207.*(t631-t885+t1132-t2224).*2.2e-4;
et1865 = t8.*t2074.*(t884+t1578-t2180+t14.*(t639-t1128-t2181+dq5.*t13.*(t86-t652))).*(-2.2e-4);
et1866 = t3293+t3537+t3542-t3316.*(t1386+t7.*(t88-t617)).*1.59e-2+t1489.*(t8.*(t92-t663)+t15.*(t621-t864)).*2.900000000000001e-4+t8.*t3411;
et1867 = t8.*t3627.*(-2.900000000000001e-4)+t8.*t3646+t2139.*t2627.*2.900000000000001e-4;
et1868 = t2000.*t3618.*2.2e-4+t2035.*t3619.*2.2e-4;
et1869 = t2576.*t3315.*2.900000000000001e-4-t3336.*(t621-t864).*2.2e-4;
et1870 = t8.*(t8.*(t92-t663)+t15.*(t621-t864)).*(t631-t885+t1132-t2224).*2.900000000000001e-4+t15.*t1207.*(t631-t885+t1132-t2224).*1.59e-2;
et1871 = t15.*t2074.*(t884+t1578-t2180+t14.*(t639-t1128-t2181+dq5.*t13.*(t86-t652))).*1.59e-2;
et1872 = t8.*t2627.*(t884+t1578-t2180+t14.*(t639-t1128-t2181+dq5.*t13.*(t86-t652))).*2.900000000000001e-4-dq7.*t8.*t1329.*7.950000000000001e-3;
et1873 = dq7.*t8.*t2058.*(-7.950000000000001e-3)-dq7.*t8.*t2108.*7.950000000000001e-3;
et1874 = dq7.*t15.*t2576.*(t1386+t7.*(t88-t617)).*(-2.900000000000001e-4);
et1875 = t3821.*(t621.*1.9738e-1-t864.*1.9738e-1-t8.*t1207.*3.466000000000001e-2+t15.*t1207.*2.324e-2);
et1876 = 3.5432e-1;
et1877 = t3288+t3535+t3538-t3316.*(t1386+t7.*(t88-t617)).*4.400000000000001e-4+t1489.*(t8.*(t92-t663)+t15.*(t621-t864)).*2.9e-4;
et1878 = t8.*t3365.*(-2.9e-4)-t8.*t3627.*2.9e-4;
et1879 = t2139.*t2627.*2.9e-4+t2000.*t3618.*1.089e-2;
et1880 = t2035.*t3619.*1.089e-2+t2576.*t3315.*2.9e-4;
et1881 = t3336.*(t621-t864).*(-1.089e-2)+t8.*(t8.*(t92-t663)+t15.*(t621-t864)).*(t631-t885+t1132-t2224).*2.9e-4;
et1882 = t15.*t1207.*(t631-t885+t1132-t2224).*4.400000000000001e-4+t15.*t2074.*(t884+t1578-t2180+t14.*(t639-t1128-t2181+dq5.*t13.*(t86-t652))).*4.400000000000001e-4;
et1883 = t8.*t2627.*(t884+t1578-t2180+t14.*(t639-t1128-t2181+dq5.*t13.*(t86-t652))).*2.9e-4+t8.*t3617.*(t1386+t7.*(t88-t617)).*2.9e-4;
et1884 = dq7.*t8.*t1329.*(-2.2e-4)-dq7.*t8.*t2058.*2.2e-4;
et1885 = dq7.*t8.*t2108.*(-2.2e-4)-dq7.*t15.*t2576.*(t1386+t7.*(t88-t617)).*2.9e-4;
et1886 = -t3291+t3365.*2.900000000000001e-4+t3527+t3642+t3654-t3662-t3665+t2654.*(t884+t1578-t2180+t14.*(t639-t1128-t2181+dq5.*t13.*(t86-t652))).*2.9e-4;
et1887 = t3336.*(t8.*(t92-t663)+t15.*(t621-t864)).*2.94e-3;
et1888 = t3845.*(t15.*t1329+t15.*t2058+t15.*t2108).*(-1.0./2.0)-((t3112+t3421+t3424+t2000.*t3618+t2035.*t3619-t3336.*(t621-t864)).*(et1767+et1768))./2.0+(t3818.*(t2035.*(t878-t1582+t2184+t7.*(t639-t1128-t2181+dq5.*t13.*(t86-t652)))+t2074.*(t884+t1578-t2180+t14.*(t639-t1128-t2181+dq5.*t13.*(t86-t652)))-t3312.*(t1386+t7.*(t88-t617))+t1207.*(t631-t885+t1132-t2224)-t2000.*(t1487+t2219-t2864+dq6.*t7.*(t88-t617))+(t621-t864).*(t642+t896-t1137-t2220)))./2.0-(t3838.*(et1769+et1770+et1771+et1772+et1773))./2.0;
et1889 = t3843.*(t2000.*t2601+t2035.*t2654-(t1529+t15.*(t92-t663)).*(t621-t864)).*(-1.0./2.0)-((t3502+t3544-t3547+t2972.*(t621-t864)+t2196.*(t642+t896-t1137-t2220)+t2816.*(t1487+t2219-t2864+dq6.*t7.*(t88-t617))).*(et1774+et1775+et1776))./2.0+((t3377+t2074.*(t878-t1582+t2184+t7.*(t639-t1128-t2181+dq5.*t13.*(t86-t652)))+t1207.*(t642+t896-t1137-t2220)).*(et1777+et1778+et1779+et1780+et1781))./2.0+et1782.*et1783+((-t2961+t3358+t3312.*(t653-t838)).*(et1784+et1785+et1786+et1787+et1788))./2.0;
et1890 = t3844.*(-t8.*t2576.*(t1386+t7.*(t88-t617))+t8.*t1207.*(t8.*(t92-t663)+t15.*(t621-t864))+t8.*t2074.*t2627).*(-1.0./2.0)-t3833.*(et1789+et1790).*3.5432e-1-(t3818.*(t2074.*(t884+t1578-t2180+t14.*(t639-t1128-t2181+dq5.*t13.*(t86-t652))).*2.0-t3312.*(t1386+t7.*(t88-t617)).*2.0+t1207.*(t631-t885+t1132-t2224).*2.0))./2.0-((t2960+t3356+t3361+t3610).*(et1791+et1792))./2.0-((t3377+t2074.*(t878-t1582+t2184+t7.*(t639-t1128-t2181+dq5.*t13.*(t86-t652)))+t1207.*(t642+t896-t1137-t2220)).*(et1793+et1794+et1795))./2.0;
et1891 = t3828.*(et1796+et1797+et1798).*(-1.0./2.0)+((-t3113+t3418+t2654.*(t884+t1578-t2180+t14.*(t639-t1128-t2181+dq5.*t13.*(t86-t652)))).*(et1799+et1800+et1801+et1802+et1803+et1804+et1805+et1806))./2.0+((t15.*t3366+t15.*t3625+t15.*t3626+t2576.*t3382+(t8.*(t92-t663)+t15.*(t621-t864)).*(t1489+t8.*(t631-t885+t1132-t2224))+t2627.*(t2139+t8.*(t884+t1578-t2180+t14.*(t639-t1128-t2181+dq5.*t13.*(t86-t652))))).*(et1807+et1808))./2.0-(t3839.*(et1809+et1810+et1811+et1812+et1813))./2.0-(t3789.*(et1814+et1815+et1816+et1817+et1818+et1819+et1820+et1821+et1822))./2.0;
et1892 = t3841.*(t2035.*(t614+t13.*(t86-t652))+t2000.*(t653-t838)-(t92-t663).*(t621-t864)).*(-1.0./2.0)-((et1823+et1824+et1825).*(t3140+t3489+t3720+t2832.*(t884+t1578-t2180+t14.*(t639-t1128-t2181+dq5.*t13.*(t86-t652)))+t3436.*(t92-t663)+t3685.*(t653-t838)))./2.0-(t3840.*(t1329+t2058+t2108))./2.0-((-t2961+t3358+t3312.*(t653-t838)).*(et1826+et1827+et1828))./2.0+((t3112+t3421+t3424+t3315.*(t1386+t7.*(t88-t617))+t2074.*t3321-t8.*t1207.*(t631-t885+t1132-t2224)).*(et1829+et1830))./2.0+(t3610.*(et1831+et1832+et1833+et1834+et1835))./2.0;
et1893 = (t3384.*(t1386+t7.*(t88-t617))+t1207.*t3039+t2074.*t3386-t2000.*t3617-t2035.*t3620-(t621-t864).*(t958-t2263+dq7.*t1601+t15.*(t642+t896-t1137-t2220))).*(et1836+et1837).*(-1.0./2.0)-(t3829.*(et1838+et1839+et1840+et1841+et1842))./2.0+((t3316.*(t1386+t7.*(t88-t617)).*2.0-t15.*t1207.*(t631-t885+t1132-t2224).*2.0-t15.*t2074.*(t884+t1578-t2180+t14.*(t639-t1128-t2181+dq5.*t13.*(t86-t652))).*2.0+dq7.*t8.*t1329+dq7.*t8.*t2058+dq7.*t8.*t2108).*(et1843+et1844))./2.0+(t3610.*(et1845+et1846))./2.0+((t2960+t3356+t3361).*(et1847+et1848))./2.0+(t3789.*(et1849+et1850+et1851+et1852+et1853+et1854+et1855+et1856+et1857))./2.0;
et1894 = t3790.*(t616.*4.9e-4-t621.*2.019e-2+t864.*2.019e-2+t870.*4.9e-4).*(-3.38795);
et1895 = t3823.*(t860.*(-4.9e-4)+t863.*2.019e-2+t1515.*2.019e-2+t1526.*4.9e-4).*(-3.38795);
et1896 = (t3782.*(et1858+et1859+et1860+et1861+et1862+et1863+et1864+et1865))./2.0-(t3782.*(et1866+et1867+et1868+et1869+et1870+et1871+et1872+et1873+et1874))./2.0+et1875.*et1876;
et1897 = t3835.*(t863.*1.9738e-1+t1515.*1.9738e-1-t8.*t2074.*3.466000000000001e-2+t15.*t2074.*2.324e-2).*3.5432e-1;
et1898 = (t3820.*(t2816.*(t1386+t7.*(t88-t617))+t1207.*t2196-t2074.*t2832))./2.0-((-t3113+t3418+t2654.*(t884+t1578-t2180+t14.*(t639-t1128-t2181+dq5.*t13.*(t86-t652)))).*(et1877+et1878+et1879+et1880+et1881+et1882+et1883+et1884+et1885))./2.0-((t1489.*(t8.*(t92-t663)+t15.*(t621-t864))+t8.*t3359-t8.*t3627+t2119.*t2576+t2139.*t2627+t2576.*t3315+t8.*(t8.*(t92-t663)+t15.*(t621-t864)).*(t631-t885+t1132-t2224)+t8.*t2627.*(t884+t1578-t2180+t14.*(t639-t1128-t2181+dq5.*t13.*(t86-t652)))+t8.*t3617.*(t1386+t7.*(t88-t617))).*(et1886+et1887))./2.0;
et1899 = t3414+t3643+t3651+t2627.*(t884+t1578-t2180+t14.*(t639-t1128-t2181+dq5.*t13.*(t86-t652))).*2.9e-4+t3336.*(t1529+t15.*(t92-t663)).*2.94e-3;
et1900 = t2576.*t3312.*2.9e-4+t2576.*t3617.*2.94e-3;
et1901 = t2601.*t3618.*2.94e-3+t2627.*t3620.*2.94e-3;
et1902 = t2654.*t3619.*2.94e-3+(t8.*(t92-t663)+t15.*(t621-t864)).*(t958-t2263+dq7.*t1601+t15.*(t642+t896-t1137-t2220)).*2.94e-3;
et1903 = (t8.*(t92-t663)+t15.*(t621-t864)).*(t631-t885+t1132-t2224).*2.9e-4;
et1904 = -t3291+t3365.*2.900000000000001e-4+t3527+t3642+t3654-t3662-t3665+t2654.*(t884+t1578-t2180+t14.*(t639-t1128-t2181+dq5.*t13.*(t86-t652))).*2.9e-4;
et1905 = t3336.*(t8.*(t92-t663)+t15.*(t621-t864)).*2.94e-3;
et1906 = t3821.*(t1601.*2.324e-2+t8.*(t92-t663).*3.466000000000001e-2-t15.*(t92-t663).*2.324e-2+t15.*(t621-t864).*3.466000000000001e-2);
et1907 = 3.5432e-1;
et1908 = -t3294+t3365.*7.950000000000001e-3+t3528+t3648+t3658-t3660-t3663+t2654.*(t884+t1578-t2180+t14.*(t639-t1128-t2181+dq5.*t13.*(t86-t652))).*2.2e-4;
et1909 = t3336.*(t8.*(t92-t663)+t15.*(t621-t864)).*2.900000000000001e-4;
et1910 = t3113.*(-2.900000000000001e-4)+t3414+t3418.*2.900000000000001e-4+t3643+t3651;
et1911 = t2654.*(t884+t1578-t2180+t14.*(t639-t1128-t2181+dq5.*t13.*(t86-t652))).*2.900000000000001e-4+t2576.*t3617.*5.88e-3;
et1912 = t2627.*t3620.*5.88e-3+(t8.*(t92-t663)+t15.*(t621-t864)).*(t958-t2263+dq7.*t1601+t15.*(t642+t896-t1137-t2220)).*5.88e-3;
et1913 = t2109.*2.94e-3+t2604.*2.94e-3;
et1914 = t2656.*2.94e-3+t1207.*(t1529+t15.*(t92-t663)).*2.900000000000001e-4;
et1915 = t2601.*(t1386+t7.*(t88-t617)).*2.900000000000001e-4-t2074.*t2654.*2.900000000000001e-4;
et1916 = t3835.*(t1635.*2.324e-2+t2080.*2.324e-2+t2081.*3.466000000000001e-2-t8.*(t614+t13.*(t86-t652)).*3.466000000000001e-2);
et1917 = 3.5432e-1;
et1918 = t3113.*(-7.950000000000001e-3)+t3417+t3418.*7.950000000000001e-3+t3649+t3653;
et1919 = t2654.*(t884+t1578-t2180+t14.*(t639-t1128-t2181+dq5.*t13.*(t86-t652))).*7.950000000000001e-3+t2576.*t3617.*5.800000000000002e-4;
et1920 = t2627.*t3620.*5.800000000000002e-4+(t8.*(t92-t663)+t15.*(t621-t864)).*(t958-t2263+dq7.*t1601+t15.*(t642+t896-t1137-t2220)).*5.800000000000002e-4;
et1921 = t2109.*2.900000000000001e-4+t2604.*2.900000000000001e-4;
et1922 = t2656.*2.900000000000001e-4+t1207.*(t1529+t15.*(t92-t663)).*7.950000000000001e-3;
et1923 = t2601.*(t1386+t7.*(t88-t617)).*7.950000000000001e-3-t2074.*t2654.*7.950000000000001e-3;
et1924 = t2109.*2.9e-4+t2604.*2.9e-4;
et1925 = t2656.*2.9e-4+t1207.*(t1529+t15.*(t92-t663)).*2.2e-4;
et1926 = t2601.*(t1386+t7.*(t88-t617)).*2.2e-4-t2074.*t2654.*2.2e-4;
et1927 = -t3294+t3365.*7.950000000000001e-3+t3528+t3648+t3658-t3660-t3663+t2654.*(t884+t1578-t2180+t14.*(t639-t1128-t2181+dq5.*t13.*(t86-t652))).*2.2e-4;
et1928 = t3336.*(t8.*(t92-t663)+t15.*(t621-t864)).*2.900000000000001e-4;
et1929 = -t3289+t3365.*2.2e-4+t3526+t3644+t3655-t3661-t3664+t2654.*(t884+t1578-t2180+t14.*(t639-t1128-t2181+dq5.*t13.*(t86-t652))).*1.089e-2;
et1930 = t3336.*(t8.*(t92-t663)+t15.*(t621-t864)).*2.9e-4;
et1931 = t3417+t3649+t3653+t2627.*(t884+t1578-t2180+t14.*(t639-t1128-t2181+dq5.*t13.*(t86-t652))).*2.2e-4+t3336.*(t1529+t15.*(t92-t663)).*2.900000000000001e-4;
et1932 = t2576.*t3312.*2.2e-4+t2576.*t3617.*2.900000000000001e-4;
et1933 = t2601.*t3618.*2.900000000000001e-4+t2627.*t3620.*2.900000000000001e-4;
et1934 = t2654.*t3619.*2.900000000000001e-4+(t8.*(t92-t663)+t15.*(t621-t864)).*(t958-t2263+dq7.*t1601+t15.*(t642+t896-t1137-t2220)).*2.900000000000001e-4;
et1935 = (t8.*(t92-t663)+t15.*(t621-t864)).*(t631-t885+t1132-t2224).*2.2e-4;
et1936 = -t3291+t3365.*2.900000000000001e-4+t3527+t3642+t3654-t3662-t3665+t2654.*(t884+t1578-t2180+t14.*(t639-t1128-t2181+dq5.*t13.*(t86-t652))).*2.9e-4;
et1937 = t3336.*(t8.*(t92-t663)+t15.*(t621-t864)).*2.94e-3;
et1938 = t3413+t3645+t3652+t2627.*(t884+t1578-t2180+t14.*(t639-t1128-t2181+dq5.*t13.*(t86-t652))).*1.089e-2+t3336.*(t1529+t15.*(t92-t663)).*2.9e-4;
et1939 = t2576.*t3312.*1.089e-2+t2576.*t3617.*2.9e-4;
et1940 = t2601.*t3618.*2.9e-4+t2627.*t3620.*2.9e-4;
et1941 = t2654.*t3619.*2.9e-4+(t8.*(t92-t663)+t15.*(t621-t864)).*(t958-t2263+dq7.*t1601+t15.*(t642+t896-t1137-t2220)).*2.9e-4;
et1942 = (t8.*(t92-t663)+t15.*(t621-t864)).*(t631-t885+t1132-t2224).*1.089e-2;
et1943 = -t3294+t3413+t3528+t3645+t3652+t2654.*(t884+t1578-t2180+t14.*(t639-t1128-t2181+dq5.*t13.*(t86-t652))).*2.2e-4+t2576.*t3617.*5.800000000000001e-4;
et1944 = t2627.*t3620.*5.800000000000001e-4+(t8.*(t92-t663)+t15.*(t621-t864)).*(t958-t2263+dq7.*t1601+t15.*(t642+t896-t1137-t2220)).*5.800000000000001e-4;
et1945 = t3789.*(et1899+et1900+et1901+et1902+et1903).*(-1.0./2.0)-((t2576.*t3617.*2.0+t2627.*t3620.*2.0+(t8.*(t92-t663)+t15.*(t621-t864)).*(t958-t2263+dq7.*t1601+t15.*(t642+t896-t1137-t2220)).*2.0).*(et1904+et1905))./2.0+et1906.*et1907-((t3360-t3626+t3618.*(t1386+t7.*(t88-t617))).*(et1908+et1909))./2.0+(t3789.*(et1910+et1911+et1912))./2.0+(t3839.*(et1913+et1914+et1915))./2.0+et1916.*et1917-(t3782.*(et1918+et1919+et1920))./2.0+(t3838.*(et1921+et1922+et1923))./2.0+(t3844.*(t2109+t2604+t2656))./2.0+(t3829.*(et1924+et1925+et1926))./2.0+((t3360-t3626+t3751+t3618.*(t1386+t7.*(t88-t617))).*(et1927+et1928))./2.0;
et1946 = ((t2627.*(t884+t1578-t2180+t14.*(t639-t1128-t2181+dq5.*t13.*(t86-t652)))+t2576.*t3312+(t8.*(t92-t663)+t15.*(t621-t864)).*(t631-t885+t1132-t2224)).*(et1929+et1930))./2.0+(t3845.*(t1207.*(t1529+t15.*(t92-t663))+t2601.*(t1386+t7.*(t88-t617))-t2074.*t2654))./2.0+(t3782.*(et1931+et1932+et1933+et1934+et1935))./2.0+((t3336.*(t1529+t15.*(t92-t663))+t2576.*t3617+t2601.*t3618+t2627.*t3620+t2654.*t3619+(t8.*(t92-t663)+t15.*(t621-t864)).*(t958-t2263+dq7.*t1601+t15.*(t642+t896-t1137-t2220))).*(et1936+et1937))./2.0;
et1947 = t3833.*(t1604.*2.324e-2+t2044.*2.324e-2+t2046.*3.466000000000001e-2-t8.*(t653-t838).*3.466000000000001e-2).*(-3.5432e-1);
et1948 = ((-t3113+t3418+t2654.*(t884+t1578-t2180+t14.*(t639-t1128-t2181+dq5.*t13.*(t86-t652)))).*(et1938+et1939+et1940+et1941+et1942))./2.0-((-t3113+t3418+t2654.*(t884+t1578-t2180+t14.*(t639-t1128-t2181+dq5.*t13.*(t86-t652)))).*(et1943+et1944))./2.0;
C = [et217+et218+et219+et220+et221+et222+et223+et224+et225+et226+et227+et228+et229;et685+et686+et687+et688+et689+et690+et691+et692+et693+et694+et695+et696+et697+et698+et699+et700+et701+et702+et703+et704+et705+et706+et707+et708+et709+et710+et711+et712+et713+et714+et715+et716;et1138+et1139+et1140+et1141+et1142+et1143+et1144+et1145+et1146+et1147+et1148+et1149+et1150+et1151+et1152+et1153+et1154+et1155+et1156+et1157+et1158+et1159+et1160+et1161+et1162+et1163+et1164+et1165+et1166+et1167+et1168;et1490+et1491+et1492+et1493+et1494+et1495+et1496+et1497+et1498+et1499+et1500+et1501+et1502+et1503+et1504+et1505+et1506+et1507+et1508+et1509+et1510+et1511+et1512+et1513+et1514+et1515+et1516+et1517;et1750+et1751+et1752+et1753+et1754+et1755+et1756+et1757+et1758+et1759+et1760+et1761+et1762+et1763+et1764+et1765+et1766;et1888+et1889+et1890+et1891+et1892+et1893+et1894+et1895+et1896+et1897+et1898;et1945+et1946+et1947+et1948];
end
